simulink model "ScriptDemo"  (R2022b)
settings: configuration reference "TmVcThermal_Configuration_sub" (kept outside this file)
undefined symbols (not defined in the file or in its folder): aaaa, bbbb, cTmComprCtrl_D_u8HvacFlowTable_db, cTmComprCtrl_D_u8HvacFlowTable_sw, cTmComprCtrl_n_i16ChillCmpIMax, cTmComprCtrl_n_i16ChillCmpIMin, cTmComprCtrl_n_i16ChillCmpIMin666, cTmComprCtrl_n_i16ChillCmpPMax, cTmComprCtrl_n_i16ChillCmpPMin, cTmComprCtrl_n_i16CmpChillCoolRpmKiMax, cTmComprCtrl_n_i16CmpChillCoolRpmKiMin, cTmComprCtrl_n_i16CmpChillCoolRpmKpMax, cTmComprCtrl_n_i16CmpChillCoolRpmKpMin, cTmComprCtrl_n_i16CmpCoolRpmKiMax, cTmComprCtrl_n_i16CmpCoolRpmKiMin, cTmComprCtrl_n_i16CmpCoolRpmKpMax, cTmComprCtrl_n_i16CmpCoolRpmKpMin, cTmComprCtrl_n_i16SM4CmpHeatKiMax, cTmComprCtrl_n_i16SM4CmpHeatKiMin, cTmComprCtrl_n_i16SM4CmpHeatKpMax, cTmComprCtrl_n_i16SM4CmpHeatKpMin, cTmComprCtrl_n_i16SM5CmpHeatKiMax, cTmComprCtrl_n_i16SM5CmpHeatKiMin, cTmComprCtrl_n_i16SM5CmpHeatKpMax, cTmComprCtrl_n_i16SM5CmpHeatKpMin, cTmComprCtrl_n_i16SM6CmpHeatKiMax, cTmComprCtrl_n_i16SM6CmpHeatKiMin, cTmComprCtrl_n_i16SM6CmpHeatKpMax, cTmComprCtrl_n_i16SM6CmpHeatKpMin, cTmComprCtrl_n_u16CmpMaxSpdFanFltLimt, cTmComprCtrl_n_u16CmpMaxSpdLoSidePFltLimt, cTmComprCtrl_n_u16CmpMaxSpdSensorFltLimt, cTmComprCtrl_n_u16CompMinRpm, cTmComprCtrl_n_u16CompRpmIncThres, cTmComprCtrl_t_u16BattCooltFFPeriod, cTmComprCtrl_t_u16BattCooltPIPeriod, cTmComprCtrl_t_u16CmpCoolFFPeriod, cTmComprCtrl_t_u16CmpCoolPIPeriod, cTmComprCtrl_t_u16CoolCmpChillFFPeriod, cTmComprCtrl_t_u16CoolCmpChillPIPeriod, cTmComprCtrl_t_u16SM4CmpHeatFFPeriod, cTmComprCtrl_t_u16SM4CmpHeatPIPeriod, cTmComprCtrl_t_u16SM5CmpHeatFFPeriod, cTmComprCtrl_t_u16SM5CmpHeatPIPeriod, cTmComprCtrl_t_u16SM6CmpHeatFFPeriod, cTmComprCtrl_t_u16SM6CmpHeatPIPeriod, cTmComprCtrl_Te_EvapClearInteg, cTmComprCtrl_Te_i16HpReqTempSaturoffset, cTmComprCtrl_Te_i16SatLpReplaceDiff, cTmComprCtrl_Te_i16SM3BatDiffStartEvapDecOffset, cTmComprCtrl_Te_i16SM3EvapLo, cTmComprCtrl_Te_i16SM3TBatDiffEntEvapDecOffset, cTmComprCtrl_Te_i16SM3TBatDiffEntEvapDecOffsetQuit, cTmComprCtrl_Te_s32ErrCmpChillPIContinueCoolH, cTmComprCtrl_Te_s32ErrCmpChillPIContinueCoolL, cTmComprCtrl_Te_s32ErrCmpPIContinueChillH, cTmComprCtrl_Te_s32ErrCmpPIContinueChillL, cTmComprCtrl_Te_s32ErrCmpPIContinueCoolH, cTmComprCtrl_Te_s32ErrCmpPIContinueCoolL, cTmComprCtrl_Te_s32ErrCmpPIContinueHeatH ... (+398)
libraries: simulink x846, PCMULib x711, simulink_need_slupdate x4
(part 5 of 49)

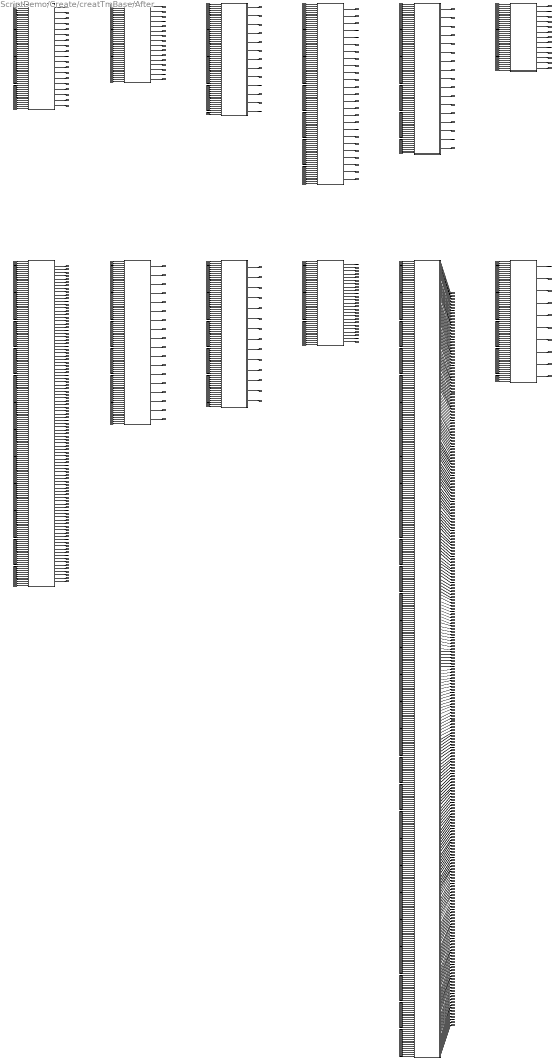
== system ScriptDemo/Create/creatTmBase/After ==
  TmAfCtrl : ModelReference  ModelNameDialog=TmAfCtrl  ScheduleRates=on  ModelReferenceVersion=13.542
  TmColtModeMgr : ModelReference  ModelNameDialog=TmColtModeMgr  ScheduleRates=on  ModelReferenceVersion=3.463
  TmColtVlvCtrl : ModelReference  ModelNameDialog=TmColtVlvCtrl  ScheduleRates=on  ModelReferenceVersion=1.683
  TmComprCtrl : ModelReference  ModelNameDialog=TmComprCtrl  ScheduleRates=on  ModelReferenceVersion=1.3185
  TmDiag : ModelReference  ModelNameDialog=TmDiag  ScheduleRates=on  ModelReferenceVersion=13.625
  TmEnergyMgr : ModelReference  ModelNameDialog=TmEnergyMgr  ScheduleRates=on  ModelReferenceVersion=1.192
  TmHvchCtrl : ModelReference  ModelNameDialog=TmHvchCtrl  ScheduleRates=on  ModelReferenceVersion=3.667
  TmPumpCtrl : ModelReference  ModelNameDialog=TmPumpCtrl  ScheduleRates=on  ModelReferenceVersion=1.672
  TmRefriModeMgr : ModelReference  ModelNameDialog=TmRefriModeMgr  ScheduleRates=on  ModelReferenceVersion=6.965
  TmRefriVlvCtrl : ModelReference  ModelNameDialog=TmRefriVlvCtrl  ScheduleRates=on  ModelReferenceVersion=1.1331
  TmSigProces : ModelReference  ModelNameDialog=TmSigProces  ScheduleRates=on  ModelReferenceVersion=1.556
  TmSovCtrl : ModelReference  ModelNameDialog=TmSovCtrl  ScheduleRates=on  ModelReferenceVersion=1.508
  wires:
  [TmRefriModeMgr_100] -> TmRefriModeMgr/1
  [yTmIn_B_AirCondEnbl] -> TmRefriModeMgr/2
  [yTmIn_B_HvacHeatgReq] -> TmRefriModeMgr/3
  [sTmIn_D_u8HvacFanSts] -> TmRefriModeMgr/4
  [sTmSigProces_Te_s32TAmb] -> TmRefriModeMgr/5
  [sTmSigProces_Te_s32HvBattCooltTOutFilter] -> TmRefriModeMgr/6
  [sTmSigProces_Te_s32BattHvMinFilter] -> TmRefriModeMgr/7
  [sTmSigProces_Te_s32EvapFanReqRamp] -> TmRefriModeMgr/8
  [sTmSigProces_Te_s32HeatrAirTReqRamp] -> TmRefriModeMgr/9
  [sTmSigProces_Te_s32HvBattCooltTFilter] -> TmRefriModeMgr/10
  [sTmDiag_D_u8BattPmpFltSt] -> TmRefriModeMgr/11
  [sTmSigProces_D_u8PowerFault] -> TmRefriModeMgr/12
  [yTmIn_B_CPSRFbSt] -> TmRefriModeMgr/13
  [sTmIn_D_u8HvActvSts] -> TmRefriModeMgr/14
  [sTmSigProces_D_u8BattThermReq] -> TmRefriModeMgr/15
  [sTmDiag_D_u8RefriMod2FInhitReq] -> TmRefriModeMgr/16
  [sTmIn_X_s32BexvPosSts] -> TmRefriModeMgr/17
  [sTmIn_n_s32ElacCmprActl] -> TmRefriModeMgr/18
  [sTmSigProces_D_u8HeatPumpConfig] -> TmRefriModeMgr/19
  [sTmComprCtrl_n_u16CompMaxRpm] -> TmRefriModeMgr/20
  [sTmSigProces_Te_s32HvacHexAirTFilter] -> TmRefriModeMgr/21
  [sTmSigProces_D_u8TempDualFlag] -> TmRefriModeMgr/22
  [sTmIn_Pw_s32HvHeatrPwrCns] -> TmRefriModeMgr/23
  [sTmColtModeMgr_D_u8WSMCurMode] -> TmRefriModeMgr/24
  [sTmSigProces_Te_s32SatLp] -> TmRefriModeMgr/25
  [sTmSigProces_md_u16BlwCool] -> TmRefriModeMgr/26
  [sTmSigProces_p_u16PLowSide] -> TmRefriModeMgr/27
  [sTmSigProces_Pw_i16ReqPwrForHeat] -> TmRefriModeMgr/28
  [sTmSigProces_Te_s32EvapFanFilter] -> TmRefriModeMgr/29
  [sTmSigProces_Te_s32TempInlet] -> TmRefriModeMgr/30
  [yTmHvchCtrl_B_HpcPtcEnad] -> TmRefriModeMgr/31
  [sTmRefriVlvCtrl_Z_u8BEXVInitState] -> TmRefriModeMgr/32
  [sTmRefriVlvCtrl_Z_u8EEXVInitState] -> TmRefriModeMgr/33
  [sTmRefriVlvCtrl_Z_u8CEXVInitState] -> TmRefriModeMgr/34
  [sTmComprCtrl_D_u8CmprRefriSwitchSt] -> TmRefriModeMgr/35
  [sTmRefriVlvCtrl_D_u8EexvRefriSwitchSt] -> TmRefriModeMgr/36
  [sTmRefriVlvCtrl_D_u8CexvRefriSwitchSt] -> TmRefriModeMgr/37
  [sTmRefriVlvCtrl_D_u8BexvRefriSwitchSt] -> TmRefriModeMgr/38
  [sTmSovCtrl_D_u8SOV1RefriSwitchSt] -> TmRefriModeMgr/39
  [sTmSovCtrl_D_u8SOV2RefriSwitchSt] -> TmRefriModeMgr/40
  [sTmSovCtrl_D_u8SOV3RefriSwitchSt] -> TmRefriModeMgr/41
  [sTmSigProces_D_u8CarChrgMode] -> TmRefriModeMgr/42
  [sTmIn_Te_s32HvBattCooltTReq] -> TmRefriModeMgr/43
  [yTmComprCtrl_B_CompOnReq] -> TmRefriModeMgr/44
  [sTmSigProces_Te_s32SatHp] -> TmRefriModeMgr/45
  [sTmIn_Te_s32WtrTInOutl] -> TmRefriModeMgr/46
  [sTmSigProces_Te_s32BattHvMaxFilter] -> TmRefriModeMgr/47
  [sTmIn_X_s32BctvPosSts] -> TmRefriModeMgr/48
  [sTmSigProces_md_u16BlwHeat] -> TmRefriModeMgr/49
  [yTmIn_B_EcoClimaSts] -> TmRefriModeMgr/50
  [sTmIn_D_u8UsgModSts1WdSts] -> TmRefriModeMgr/51
  [sTmIn_X_s32ClimtRcirc] -> TmRefriModeMgr/52
  [sTmColtModeMgr_B_HvBattClntHtgHvac] -> TmRefriModeMgr/53
  [sTmIn_Te_s32HvBattTAvg] -> TmRefriModeMgr/54
  [sTmHvchCtrl_Te_s32CabinPtcTempReq] -> TmRefriModeMgr/55
  TmRefriModeMgr/1 -> [sTmRefriModeMgr_D_u8CabinCoolReq]
  TmRefriModeMgr/2 -> [sTmRefriModeMgr_D_u8CabinHeatReq]
  TmRefriModeMgr/3 -> [sTmRefriModeMgr_D_u8BatCoolReq]
  TmRefriModeMgr/4 -> [sTmRefriModeMgr_D_u8HPAbleToWHRFlag]
  TmRefriModeMgr/5 -> [sTmRefriModeMgr_D_u8ModeStatus]
  TmRefriModeMgr/6 -> [sTmRefriModeMgr_D_u8HPCurMode]
  TmRefriModeMgr/7 -> [sTmRefriModeMgr_D_u8HpModeMainState]
  TmRefriModeMgr/8 -> [sTmRefriModeMgr_D_u8HpModeCmd]
  TmRefriModeMgr/9 -> [sTmRefriModeMgr_D_u8HpFmCmd]
  TmRefriModeMgr/10 -> [sTmRefriModeMgr_D_u8HpReqPTCState]
  TmRefriModeMgr/11 -> [yTmRefriModeMgr_B_InterChillDeicing]
  TmRefriModeMgr/12 -> [yTmRefriModeMgr_B_DeicePTCReq]
  TmRefriModeMgr/13 -> [yTmRefriModeMgr_B_CoolOCRMode]
  TmRefriModeMgr/14 -> [yTmRefriModeMgr_B_NeedPTCInOCR]
  TmRefriModeMgr/15 -> [yTmRefriModeMgr_B_CoolModeInCycle]
  TmRefriModeMgr/16 -> [sTmRefriModeMgr_D_u8ModeSwitchType]
  TmRefriModeMgr/17 -> [sTmRefriModeMgr_D_u8HvacMixClapOpenReq]
  TmRefriModeMgr/18 -> [yTmRefriModeMgr_B_HpReqPTCAddHeat]
  TmRefriModeMgr/19 -> [yTmRefriModeMgr_B_HeatModeInCycle]
  [TmColtModeMgr_100] -> TmColtModeMgr/1
  [yTmIn_B_CPSRFbSt] -> TmColtModeMgr/2
  [sTmSigProces_D_u8PowerFault] -> TmColtModeMgr/3
  [yTmRefriModeMgr_B_InterChillDeicing] -> TmColtModeMgr/4
  [sTmDiag_D_u8BctvFltSt] -> TmColtModeMgr/5
  [sTmDiag_D_u8BcfvFltSt] -> TmColtModeMgr/6
  [sTmDiag_D_u8ClntTforEmCircFltSt] -> TmColtModeMgr/7
  [sTmDiag_D_u8EmPmpFltSt] -> TmColtModeMgr/8
  [sTmDiag_D_u8BattPmpFltSt] -> TmColtModeMgr/9
  [sTmIn_D_u8HvActvSts] -> TmColtModeMgr/10
  [sTmDiag_D_u8WaterMod2FInhitReq] -> TmColtModeMgr/11
  [sTmSigProces_D_u8BattThermReq] -> TmColtModeMgr/12
  [sTmIn_v_s32VehSpdLgt] -> TmColtModeMgr/13
  [sTmSigProces_Te_s32MotorCoolt] -> TmColtModeMgr/14
  [sTmSigProces_Te_s32BattHvMaxFilter] -> TmColtModeMgr/15
  [sTmSigProces_Te_s32BattHvMinFilter] -> TmColtModeMgr/16
  [sTmSigProces_D_u8PassiveCoolEnFlag] -> TmColtModeMgr/17
  [sTmSigProces_Te_s32HvBattCooltTOutFilter] -> TmColtModeMgr/18
  [yTmRefriModeMgr_B_NeedPTCInOCR] -> TmColtModeMgr/19
  [yTmRefriModeMgr_B_CoolOCRMode] -> TmColtModeMgr/20
  [sTmSigProces_Te_s32HeatrAirTReqRamp] -> TmColtModeMgr/21
  [sTmIn_X_s32BcfvPosSts] -> TmColtModeMgr/22
  [sTmIn_X_s32BctvPosSts] -> TmColtModeMgr/23
  [sTmIn_D_u8HeatPump] -> TmColtModeMgr/24
  [sTmSigProces_Te_s32TAmb] -> TmColtModeMgr/25
  [sTmIn_Te_s32HvBattTAvg] -> TmColtModeMgr/26
  [sTmRefriModeMgr_D_u8CabinHeatReq] -> TmColtModeMgr/27
  [sTmSigProces_Te_s32HvBattCooltTFilter] -> TmColtModeMgr/28
  [yTmRefriModeMgr_B_DeicePTCReq] -> TmColtModeMgr/29
  [sTmIn_D_u8HeatStopReq] -> TmColtModeMgr/30
  [yTmHvchCtrl_B_EdMoterHeatEnad] -> TmColtModeMgr/31
  [sTmComprCtrl_D_u32AcOffCode] -> TmColtModeMgr/32
  [sTmComprCtrl_D_u32AcOffCode2] -> TmColtModeMgr/33
  [sTmEnergyMgr_Pw_s32HvCoolgPwrNormDes] -> TmColtModeMgr/34
  [sTmIn_Pw_s32HvCoolgAllwd] -> TmColtModeMgr/35
  [sTmIn_Pw_s32HvHeatgAllwd] -> TmColtModeMgr/36
  [sTmHvchCtrl_D_u32PtcOffCode] -> TmColtModeMgr/37
  [sTmEnergyMgr_Pw_s32HvHeatgPwrNormDes] -> TmColtModeMgr/38
  [yTmRefriModeMgr_B_HeatModeInCycle] -> TmColtModeMgr/39
  [sTmIn_D_u8UsgModSts1WdSts] -> TmColtModeMgr/40
  [sTmRefriModeMgr_D_u8HpReqPTCState] -> TmColtModeMgr/41
  TmColtModeMgr/1 -> [sTmColtModeMgr_D_u8WSMSwitchState]
  TmColtModeMgr/2 -> [sTmColtModeMgr_D_u8WSMCurMode]
  TmColtModeMgr/3 -> [sTmColtModeMgr_D_u8WSMReqModeFront]
  TmColtModeMgr/4 -> [yTmColtModeMgr_B_BatReqForDeiceFlag]
  TmColtModeMgr/5 -> [sTmColtModeMgr_D_u8BatReqPTCState]
  TmColtModeMgr/6 -> [sTmColtModeMgr_D_u8WaterMainState]
  TmColtModeMgr/7 -> [sTmColtModeMgr_D_u8WSMReqMode]
  TmColtModeMgr/8 -> [sTmColtModeMgr_B_HvBattClntHtgHvac]
  TmColtModeMgr/9 -> [yTmColtModeMgr_B_HeatSave]
  TmColtModeMgr/10 -> [yTmColtModeMgr_B_HvEMotorBattClntHtgHvac]
  TmColtModeMgr/11 -> [yTmColtModeMgr_B_DeiceBattAddHeat]
  TmColtModeMgr/12 -> [yTmColtModeMgr_B_NeedPTCInOCR]
  TmColtModeMgr/13 -> [yTmColtModeMgr_B_EMoterHeatModEnad]
  TmColtModeMgr/14 -> [sTmColtModeMgr_D_u8WSMFunction]
  TmColtModeMgr/15 -> [yTmColtModeMgr_B_EMoterHeatModSave]
  TmColtModeMgr/16 -> [sTmColtModeMgr_D_u8HvBattThermReqFb]
  [TmHvchCtrl_100] -> TmHvchCtrl/1
  [sTmColtModeMgr_D_u8BatReqPTCState] -> TmHvchCtrl/2
  [sTmRefriModeMgr_D_u8HpReqPTCState] -> TmHvchCtrl/3
  [yTmColtModeMgr_B_DeiceBattAddHeat] -> TmHvchCtrl/4
  [yTmRefriModeMgr_B_NeedPTCInOCR] -> TmHvchCtrl/5
  [sTmDiag_D_u8WaterMod2FInhitReq] -> TmHvchCtrl/6
  [yTmIn_B_CPSRFbSt] -> TmHvchCtrl/7
  [sTmSigProces_D_u8PowerFault] -> TmHvchCtrl/8
  [sTmIn_D_u8HeatStopReq] -> TmHvchCtrl/9
  [sTmIn_D_u8HvActvSts] -> TmHvchCtrl/10
  [yTmIn_B_HvCooltHeatrEnad] -> TmHvchCtrl/11
  [sTmDiag_D_u8HvchFltSt] -> TmHvchCtrl/12
  [sTmDiag_D_u8HmPmpFltSt] -> TmHvchCtrl/13
  [sTmDiag_D_u8BattClntLvlFltSt] -> TmHvchCtrl/14
  [sTmDiag_D_u8BctvFltSt] -> TmHvchCtrl/15
  [sTmPumpCtrl_X_s32HpumpPwmReq] -> TmHvchCtrl/16
  [sTmSigProces_Te_s32HeatrAirTReqRamp] -> TmHvchCtrl/17
  [sTmIn_Te_s32HvBattCooltTReq] -> TmHvchCtrl/18
  [sTmIn_Te_s32HvacHexAirT] -> TmHvchCtrl/19
  [sTmSigProces_Te_s32TAmb] -> TmHvchCtrl/20
  [yTmIn_B_HvacHexAirTQf] -> TmHvchCtrl/21
  [sTmIn_Te_s32HvBattCooltT] -> TmHvchCtrl/22
  [sTmIn_Te_s32WtrTInIntk] -> TmHvchCtrl/23
  [sTmIn_Te_s32WtrTInOutl] -> TmHvchCtrl/24
  [sTmColtModeMgr_B_HvBattClntHtgHvac] -> TmHvchCtrl/25
  [sTmDiag_D_u8BattPmpFltSt] -> TmHvchCtrl/26
  [sTmSigProces_D_u8BattThermReq] -> TmHvchCtrl/27
  [sTmIn_X_s32BctvPosSts] -> TmHvchCtrl/28
  [sTmSigProces_md_u16BlwHeat] -> TmHvchCtrl/29
  [sTmDiag_D_u8HvBattCooltTFltSt] -> TmHvchCtrl/30
  [sTmDiag_D_u8HvBattCooltTOutFltSt] -> TmHvchCtrl/31
  [yTmIn_B_ImpactDetect] -> TmHvchCtrl/32
  [sTmIn_D_u8HeatrStsSig] -> TmHvchCtrl/33
  [yTmIn_B_EmActivHeatAllwd] -> TmHvchCtrl/34
  [sTmSigProces_D_u8HeatPumpConfig] -> TmHvchCtrl/35
  [sTmSigProces_D_u8ElecDrivelineConfig] -> TmHvchCtrl/36
  [sTmIn_D_u8IsgHeatFdBck] -> TmHvchCtrl/37
  [sTmIn_D_u8WhlMotSysHeatFdBck] -> TmHvchCtrl/38
  [sTmIn_Pw_s32IsgHeatPwrMax] -> TmHvchCtrl/39
  [sTmIn_Pw_s32WhlMotSysHeatPwrMax] -> TmHvchCtrl/40
  [sTmSigProces_Te_s32HvBattCooltTFilter] -> TmHvchCtrl/41
  [sTmIn_Pw_s32IsgHeatPwrAct] -> TmHvchCtrl/42
  [sTmIn_Pw_s32WhlMotSysHeatPwrAct] -> TmHvchCtrl/43
  [sTmSigProces_D_u8CarChrgMode] -> TmHvchCtrl/44
  [sTmSigProces_Te_s32BattHvMinFilter] -> TmHvchCtrl/45
  [sTmEnergyMgr_Pw_s32ElecDrvHeatgPwrAllwd] -> TmHvchCtrl/46
  [sTmIn_X_s32BattCooltPmpPwmFb] -> TmHvchCtrl/47
  [sTmDiag_D_u8ClntTforEmCircFltSt] -> TmHvchCtrl/48
  [yTmRefriModeMgr_B_HpReqPTCAddHeat] -> TmHvchCtrl/49
  [sTmSigProces_Te_s32EvapFanFilter] -> TmHvchCtrl/50
  [yTmColtModeMgr_B_HvEMotorBattClntHtgHvac] -> TmHvchCtrl/51
  [sTmIn_D_u8HeatPump] -> TmHvchCtrl/52
  [sTmIn_D_u8OnBdChrgrHndlSts] -> TmHvchCtrl/53
  [sTmRefriModeMgr_D_u8CabinHeatReq] -> TmHvchCtrl/54
  [sTmDiag_Te_s32PtcTReq2F] -> TmHvchCtrl/55
  [sTmDiag_D_u8PtcT2FEnaState] -> TmHvchCtrl/56
  [yTmDiag_B_PtcEnaReq2F] -> TmHvchCtrl/57
  [sTmDiag_D_u8PtcEna2FEnaState] -> TmHvchCtrl/58
  TmHvchCtrl/1 -> [yTmHvchCtrl_B_HPumpPtcStopOk]
  TmHvchCtrl/2 -> [sTmHvchCtrl_Te_s32HpcPtcTempReq]
  TmHvchCtrl/3 -> [yTmHvchCtrl_B_HpcPtcEnad]
  TmHvchCtrl/4 -> [yTmHvchCtrl_B_HvWtrHeatrActDischrgReq]
  TmHvchCtrl/5 -> [sTmHvchCtrl_D_u32PtcOffCode]
  TmHvchCtrl/6 -> [yTmHvchCtrl_B_FrntHeatModEnad]
  TmHvchCtrl/7 -> [yTmHvchCtrl_B_RearHeatModEnad]
  TmHvchCtrl/8 -> [sTmHvchCtrl_Pw_s32ElecDrvHeatgPwrReq]
  TmHvchCtrl/9 -> [sTmHvchCtrl_Pw_u16FrntHeatPwrAllwd]
  TmHvchCtrl/10 -> [sTmHvchCtrl_Pw_u16RearHeatPwrAllwd]
  TmHvchCtrl/11 -> [yTmHvchCtrl_B_EdMoterHeatEnad]
  TmHvchCtrl/12 -> [sTmHvchCtrl_Te_s32CabinPtcTempReq]
  TmHvchCtrl/13 -> [sTmHvchCtrl_D_u8PTCOffState]
  [TmComprCtrl_100] -> TmComprCtrl/1
  [sTmDiag_D_u8BexvFltSt] -> TmComprCtrl/2
  [sTmDiag_D_u8CexvFltSt] -> TmComprCtrl/3
  [sTmDiag_D_u8EexvFltSt] -> TmComprCtrl/4
  [sTmDiag_D_u8FanFltSt] -> TmComprCtrl/5
  [sTmDiag_D_u8HiSidePFltSt] -> TmComprCtrl/6
  [sTmDiag_D_u8LoSidePFltSt] -> TmComprCtrl/7
  [sTmDiag_D_u8OutrCondOutTFltSt] -> TmComprCtrl/8
  [sTmDiag_D_u8Sov1FltSt] -> TmComprCtrl/9
  [sTmDiag_D_u8Sov2FltSt] -> TmComprCtrl/10
  [sTmDiag_D_u8Sov3FltSt] -> TmComprCtrl/11
  [sTmDiag_D_u8Sov4FltSt] -> TmComprCtrl/12
  [sTmDiag_D_u8Sov5FltSt] -> TmComprCtrl/13
  [sTmDiag_D_u8TeEvapFltSt] -> TmComprCtrl/14
  [sTmIn_D_u8DCChrgSt] -> TmComprCtrl/15
  [sTmIn_D_u8HeatPump] -> TmComprCtrl/16
  [sTmIn_D_u8HvActvSts] -> TmComprCtrl/17
  [sTmIn_I_s32ElacCmprHvActl] -> TmComprCtrl/18
  [sTmIn_Pw_s32HvCoolgAllwd] -> TmComprCtrl/19
  [sTmIn_Te_s32BattHv] -> TmComprCtrl/20
  [sTmSigProces_Te_s32EvapFanReqRamp] -> TmComprCtrl/21
  [sTmIn_Te_s32HvBattCooltT] -> TmComprCtrl/22
  [sTmIn_Te_s32HvBattCooltTReq] -> TmComprCtrl/23
  [sTmIn_U_s32ElacCmprHvActl] -> TmComprCtrl/24
  [sTmIn_X_s32BexvPosSts] -> TmComprCtrl/25
  [sTmIn_X_s32CexvPosSts] -> TmComprCtrl/26
  [sTmIn_X_s32ClimtRcirc] -> TmComprCtrl/27
  [sTmIn_X_s32EexvPosSts] -> TmComprCtrl/28
  [sTmIn_X_s32HvacTFlpActlPosnFrtRowLe] -> TmComprCtrl/29
  [sTmIn_X_s32HvacTFlpActlPosnFrtRowRi] -> TmComprCtrl/30
  [sTmIn_n_s32ElacCmprActl] -> TmComprCtrl/31
  [sTmIn_v_s32VehSpdLgt] -> TmComprCtrl/32
  [sTmRefriModeMgr_D_u8HPCurMode] -> TmComprCtrl/33
  [sTmRefriModeMgr_D_u8HpFmCmd] -> TmComprCtrl/34
  [sTmRefriModeMgr_D_u8HpModeMainState] -> TmComprCtrl/35
  [sTmRefriVlvCtrl_Z_u8BEXVInitState] -> TmComprCtrl/36
  [sTmRefriVlvCtrl_Z_u8CEXVInitState] -> TmComprCtrl/37
  [sTmRefriVlvCtrl_Z_u8EEXVInitState] -> TmComprCtrl/38
  [sTmSigProces_D_u8BattThermReq] -> TmComprCtrl/39
  [sTmSigProces_D_u8HvBattCoolgReq] -> TmComprCtrl/40
  [sTmSigProces_D_u8PowerFault] -> TmComprCtrl/41
  [sTmSigProces_Te_s32CompDischarge] -> TmComprCtrl/42
  [sTmSigProces_Te_s32EvapFanFilter] -> TmComprCtrl/43
  [sTmSigProces_Te_s32HeatrAirTReqRamp] -> TmComprCtrl/44
  [sTmSigProces_Te_s32HvBattCooltTFilter] -> TmComprCtrl/45
  [sTmSigProces_Te_s32HvBattCooltTOutFilter] -> TmComprCtrl/46
  [sTmSigProces_Te_s32HvacHexAirTFilter] -> TmComprCtrl/47
  [sTmSigProces_Te_s32TempInlet] -> TmComprCtrl/48
  [sTmSigProces_Te_s32SatHp] -> TmComprCtrl/49
  [sTmSigProces_Te_s32SatLp] -> TmComprCtrl/50
  [sTmSigProces_md_u16BlwHeat] -> TmComprCtrl/51
  [sTmSigProces_p_u16PHighSide] -> TmComprCtrl/52
  [sTmSigProces_p_u16PLowSide] -> TmComprCtrl/53
  [sTmSovCtrl_D_u8HpcSov1OnOffSts] -> TmComprCtrl/54
  [sTmSovCtrl_D_u8HpcSov2OnOffSts] -> TmComprCtrl/55
  [sTmSovCtrl_D_u8HpcSov3OnOffSts] -> TmComprCtrl/56
  [sTmSovCtrl_D_u8HpcSov4OnOffSts] -> TmComprCtrl/57
  [sTmSovCtrl_D_u8HpcSov5OnOffSts] -> TmComprCtrl/58
  [yTmHvchCtrl_B_HpcPtcEnad] -> TmComprCtrl/59
  [yTmIn_B_ElAcEnable] -> TmComprCtrl/60
  [yTmRefriModeMgr_B_CoolModeInCycle] -> TmComprCtrl/61
  [yTmSovCtrl_B_HpmSov1ActvCmd] -> TmComprCtrl/62
  [yTmSovCtrl_B_HpmSov2ActvCmd] -> TmComprCtrl/63
  [yTmSovCtrl_B_HpmSov3ActvCmd] -> TmComprCtrl/64
  [yTmSovCtrl_B_HpmSov4ActvCmd] -> TmComprCtrl/65
  [yTmSovCtrl_B_HpmSov5ActvCmd] -> TmComprCtrl/66
  [sTmDiag_D_u8AccmFltSt] -> TmComprCtrl/67
  [sTmDiag_D_u8CmprPwrEna2FEnaState] -> TmComprCtrl/68
  [sTmDiag_D_u8CmprSpdEna2FEnaState] -> TmComprCtrl/69
  [sTmDiag_D_u8CmprStsEna2FEnaState] -> TmComprCtrl/70
  [sTmDiag_D_u8CmprStsEnaReq2F] -> TmComprCtrl/71
  [sTmDiag_D_u8HiSidePNHPFltSt] -> TmComprCtrl/72
  [sTmDiag_D_u8HvacHexAirTFltSt] -> TmComprCtrl/73
  [sTmDiag_D_u8InrCondOutTFltSt] -> TmComprCtrl/74
  [sTmDiag_D_u8RefrilackFltSt] -> TmComprCtrl/75
  [sTmDiag_Pw_s32CmprPwrEnaReq2F] -> TmComprCtrl/76
  [sTmDiag_n_s32CmprSpdReq2F] -> TmComprCtrl/77
  [sTmDiag_D_u8CmprDischrgTFltSt] -> TmComprCtrl/78
  [sTmSigProces_Pw_i16ReqPwrForHeat] -> TmComprCtrl/79
  [sTmSigProces_md_u16BlwCool] -> TmComprCtrl/80
  [sTmSigProces_D_u8CarChrgMode] -> TmComprCtrl/81
  [sTmIn_D_u8ElecDriveline] -> TmComprCtrl/82
  [sTmRefriModeMgr_D_u8CabinCoolReq] -> TmComprCtrl/83
  [sTmRefriModeMgr_D_u8CabinHeatReq] -> TmComprCtrl/84
  [sTmRefriModeMgr_D_u8HpModeCmd] -> TmComprCtrl/85
  [sTmSigProces_Te_s32TAmb] -> TmComprCtrl/86
  [sTmRefriModeMgr_D_u8ModeSwitchType] -> TmComprCtrl/87
  [yTmRefriModeMgr_B_CoolOCRMode] -> TmComprCtrl/88
  [sTmDiag_D_u8BattPmpFltSt] -> TmComprCtrl/89
  [sTmDiag_D_u8HvBattCooltTFltSt] -> TmComprCtrl/90
  [sTmDiag_D_u8HvBattCooltTOutFltSt] -> TmComprCtrl/91
  [sTmIn_D_u8OnBdChrgrHndlSts] -> TmComprCtrl/92
  [sTmSigProces_Pw_i16ReqPwrForCool] -> TmComprCtrl/93
  [yTmRefriModeMgr_B_HeatModeInCycle] -> TmComprCtrl/94
  TmComprCtrl/1 -> [sTmComprCtrl_D_u32AcOffCode]
  TmComprCtrl/2 -> [sTmComprCtrl_n_u16CompRpmReq]
  TmComprCtrl/3 -> [yTmComprCtrl_B_CompOnReq]
  TmComprCtrl/4 -> [sTmComprCtrl_n_u16CompMaxRpm]
  TmComprCtrl/5 -> [sTmComprCtrl_D_u8AcOffCode0]
  TmComprCtrl/6 -> [sTmComprCtrl_D_u8AcOffCode1]
  TmComprCtrl/7 -> [sTmComprCtrl_D_u8AcOffCode2]
  TmComprCtrl/8 -> [sTmComprCtrl_D_u8AcOffCode3]
  TmComprCtrl/9 -> [sTmComprCtrl_D_u8AirCondCmpsrStats]
  TmComprCtrl/10 -> [sTmComprCtrl_Pw_s32ClimaCoolgPwrCritDes]
  TmComprCtrl/11 -> [sTmComprCtrl_Pw_s32CmprPwrNormDes]
  TmComprCtrl/12 -> [sTmComprCtrl_Pw_s32CoolgPwrCritDes]
  TmComprCtrl/13 -> [sTmComprCtrl_Pw_s32ElacCmprMax]
  TmComprCtrl/14 -> [sTmComprCtrl_Pw_s32HpcHvCoolgPwrCns]
  TmComprCtrl/15 -> [sTmComprCtrl_X_u8HpcCoolgLoad]
  TmComprCtrl/16 -> [sTmComprCtrl_t_u32CmprRunTime]
  TmComprCtrl/17 -> [yTmComprCtrl_B_AcPHiSideHi]
  TmComprCtrl/18 -> [yTmComprCtrl_B_AcPLoSideLo]
  TmComprCtrl/19 -> [yTmComprCtrl_B_HpcCoolgLimd]
  TmComprCtrl/20 -> [yTmComprCtrl_B_AcPHiSideLo]
  TmComprCtrl/21 -> [sTmComprCtrl_D_u32AcOffCode2]
  TmComprCtrl/22 -> [sTmComprCtrl_D_u8AcOffCode4]
  TmComprCtrl/23 -> [sTmComprCtrl_D_u8HvacFlowLevel]
  TmComprCtrl/24 -> [sTmComprCtrl_D_u8CmprRefriSwitchSt]
  TmComprCtrl/25 -> [sTmComprCtrl_D_u8ACOffState]
  [TmRefriVlvCtrl_100] -> TmRefriVlvCtrl/1
  [sTmComprCtrl_D_u8CmprRefriSwitchSt] -> TmRefriVlvCtrl/2
  [sTmComprCtrl_D_u8HvacFlowLevel] -> TmRefriVlvCtrl/3
  [sTmComprCtrl_n_u16CompMaxRpm] -> TmRefriVlvCtrl/4
  [sTmComprCtrl_n_u16CompRpmReq] -> TmRefriVlvCtrl/5
  [sTmDiag_D_u8BexvCal2FEnaState] -> TmRefriVlvCtrl/6
  [sTmDiag_D_u8BexvFltSt] -> TmRefriVlvCtrl/7
  [sTmDiag_D_u8BexvMoveEna2FEnaState] -> TmRefriVlvCtrl/8
  [sTmDiag_D_u8BexvPosnReq2FEnaState] -> TmRefriVlvCtrl/9
  [sTmDiag_D_u8CexvCal2FEnaState] -> TmRefriVlvCtrl/10
  [sTmDiag_D_u8CexvFltSt] -> TmRefriVlvCtrl/11
  [sTmDiag_D_u8CexvMoveEna2FEnaState] -> TmRefriVlvCtrl/12
  [sTmDiag_D_u8CexvPosnReq2FEnaState] -> TmRefriVlvCtrl/13
  [sTmDiag_D_u8ChillerOutTFltSt] -> TmRefriVlvCtrl/14
  [sTmDiag_D_u8EexvCal2FEnaState] -> TmRefriVlvCtrl/15
  [sTmDiag_D_u8EexvFltSt] -> TmRefriVlvCtrl/16
  [sTmDiag_D_u8EexvMoveEna2FEnaState] -> TmRefriVlvCtrl/17
  [sTmDiag_D_u8EexvPosnReq2FEnaState] -> TmRefriVlvCtrl/18
  [sTmDiag_D_u8EvapOutTFltSt] -> TmRefriVlvCtrl/19
  [sTmDiag_D_u8HiSidePFltSt] -> TmRefriVlvCtrl/20
  [sTmDiag_D_u8InrCondOutTFltSt] -> TmRefriVlvCtrl/21
  [sTmDiag_D_u8LoSidePFltSt] -> TmRefriVlvCtrl/22
  [sTmDiag_D_u8OutrCondOutTFltSt] -> TmRefriVlvCtrl/23
  [sTmDiag_X_s32BexvPosnReq2F] -> TmRefriVlvCtrl/24
  [sTmDiag_X_s32CexvPosnReq2F] -> TmRefriVlvCtrl/25
  [sTmDiag_X_s32EexvPosnReq2F] -> TmRefriVlvCtrl/26
  [sTmIn_D_u8BexvCalibSts] -> TmRefriVlvCtrl/27
  [sTmIn_D_u8CexvCalibSts] -> TmRefriVlvCtrl/28
  [sTmIn_D_u8EexvCalibSts] -> TmRefriVlvCtrl/29
  [sTmIn_D_u8HeatPump] -> TmRefriVlvCtrl/30
  [sTmIn_D_u8HvBattCoolgReq] -> TmRefriVlvCtrl/31
  [sTmIn_L_s32HvBattCoolFlow1] -> TmRefriVlvCtrl/32
  [sTmIn_Te_s32HvBattCooltTReq] -> TmRefriVlvCtrl/33
  [sTmIn_X_s32BexvPosSts] -> TmRefriVlvCtrl/34
  [sTmIn_X_s32CexvPosSts] -> TmRefriVlvCtrl/35
  [sTmIn_X_s32EexvPosSts] -> TmRefriVlvCtrl/36
  [sTmIn_v_s32VehSpdLgt] -> TmRefriVlvCtrl/37
  [sTmRefriModeMgr_D_u8HPCurMode] -> TmRefriVlvCtrl/38
  [sTmRefriModeMgr_D_u8HpModeCmd] -> TmRefriVlvCtrl/39
  [sTmRefriModeMgr_D_u8HpModeMainState] -> TmRefriVlvCtrl/40
  [sTmRefriModeMgr_D_u8HpReqPTCState] -> TmRefriVlvCtrl/41
  [sTmRefriModeMgr_D_u8ModeSwitchType] -> TmRefriVlvCtrl/42
  [sTmSigProces_D_u8CarChrgMode] -> TmRefriVlvCtrl/43
  [sTmSigProces_D_u8LargerCoolingFlag] -> TmRefriVlvCtrl/44
  [sTmSigProces_Pw_i16ReqPwrForCool] -> TmRefriVlvCtrl/45
  [sTmSigProces_Te_s32BattHvMaxFilter] -> TmRefriVlvCtrl/46
  [sTmSigProces_Te_s32CompDischarge] -> TmRefriVlvCtrl/47
  [sTmSigProces_Te_s32CoolSH] -> TmRefriVlvCtrl/48
  [sTmSigProces_Te_s32CurInterSC] -> TmRefriVlvCtrl/49
  [sTmSigProces_Te_s32CurOutSC] -> TmRefriVlvCtrl/50
  [sTmSigProces_Te_s32CurSCCalValue] -> TmRefriVlvCtrl/51
  [sTmSigProces_Te_s32EvapFanFilter] -> TmRefriVlvCtrl/52
  [sTmSigProces_Te_s32EvapFanReqRamp] -> TmRefriVlvCtrl/53
  [sTmSigProces_Te_s32HeatSH] -> TmRefriVlvCtrl/54
  [sTmSigProces_Te_s32HeatrAirTReqRamp] -> TmRefriVlvCtrl/55
  [sTmSigProces_Te_s32HvBattCooltTFilter] -> TmRefriVlvCtrl/56
  [sTmSigProces_Te_s32HvBattCooltTOutFilter] -> TmRefriVlvCtrl/57
  [sTmSigProces_Te_s32HvacHexAirTFilter] -> TmRefriVlvCtrl/58
  [sTmSigProces_Te_s32InletCal] -> TmRefriVlvCtrl/59
  [sTmSigProces_Te_s32TAmb] -> TmRefriVlvCtrl/60
  [sTmSigProces_md_u16BlwCool] -> TmRefriVlvCtrl/61
  [sTmSigProces_md_u16BlwHeat] -> TmRefriVlvCtrl/62
  [sTmSigProces_p_u16PHighSide] -> TmRefriVlvCtrl/63
  [sTmSigProces_p_u16PLowSide] -> TmRefriVlvCtrl/64
  [sTmSovCtrl_D_u8SOV2RefriSwitchSt] -> TmRefriVlvCtrl/65
  [yTmComprCtrl_B_CompOnReq] -> TmRefriVlvCtrl/66
  [yTmDiag_B_BexvCalReq2F] -> TmRefriVlvCtrl/67
  [yTmDiag_B_BexvMoveEnReq2F] -> TmRefriVlvCtrl/68
  [yTmDiag_B_CexvCalReq2F] -> TmRefriVlvCtrl/69
  [yTmDiag_B_CexvMoveEnReq2F] -> TmRefriVlvCtrl/70
  [yTmDiag_B_EexvCalReq2F] -> TmRefriVlvCtrl/71
  [yTmDiag_B_EexvMoveEnReq2F] -> TmRefriVlvCtrl/72
  [yTmHvchCtrl_B_HpcPtcEnad] -> TmRefriVlvCtrl/73
  [yTmIn_B_CPSRFbSt] -> TmRefriVlvCtrl/74
  [yTmIn_B_HmiMaxACReq] -> TmRefriVlvCtrl/75
  [yTmRefriModeMgr_B_CoolModeInCycle] -> TmRefriVlvCtrl/76
  [yTmRefriModeMgr_B_CoolOCRMode] -> TmRefriVlvCtrl/77
  [yTmRefriModeMgr_B_InterChillDeicing] -> TmRefriVlvCtrl/78
  TmRefriVlvCtrl/1 -> [yTmRefriVlvCtrl_B_HpcCexvMovEnable]
  TmRefriVlvCtrl/2 -> [yTmRefriVlvCtrl_B_CexvCalibReq]
  TmRefriVlvCtrl/3 -> [yTmRefriVlvCtrl_B_HpcEexvMovEnable]
  TmRefriVlvCtrl/4 -> [yTmRefriVlvCtrl_B_EexvCalibReq]
  TmRefriVlvCtrl/5 -> [yTmRefriVlvCtrl_B_HpcBexvMovEnable]
  TmRefriVlvCtrl/6 -> [yTmRefriVlvCtrl_B_BexvCalibReq]
  TmRefriVlvCtrl/7 -> [sTmRefriVlvCtrl_X_s32SM3BexvMaxPos]
  TmRefriVlvCtrl/8 -> [yTmRefriVlvCtrl_B_EvapBattTLimBexvEna]
  TmRefriVlvCtrl/9 -> [sTmRefriVlvCtrl_D_u8EexvRefriSwitchSt]
  TmRefriVlvCtrl/10 -> [sTmRefriVlvCtrl_D_u8CexvRefriSwitchSt]
  TmRefriVlvCtrl/11 -> [sTmRefriVlvCtrl_D_u8BexvRefriSwitchSt]
  TmRefriVlvCtrl/12 -> [sTmRefriVlvCtrl_X_s32EEXVPosReq]
  TmRefriVlvCtrl/13 -> [sTmRefriVlvCtrl_Z_u8CEXVInitState]
  TmRefriVlvCtrl/14 -> [sTmRefriVlvCtrl_Z_u8EEXVInitState]
  TmRefriVlvCtrl/15 -> [sTmRefriVlvCtrl_Z_u8BEXVInitState]
  TmRefriVlvCtrl/16 -> [sTmRefriVlvCtrl_X_s32CEXVPosReq]
  TmRefriVlvCtrl/17 -> [sTmRefriVlvCtrl_X_s32BEXVPosReq]
  [TmSovCtrl_100] -> TmSovCtrl/1
  [sTmRefriModeMgr_D_u8HpModeMainState] -> TmSovCtrl/2
  [sTmDiag_D_u8ChillerValve2FEnState] -> TmSovCtrl/3
  [sTmDiag_D_u8EvaprVlvFrnt2FEnState] -> TmSovCtrl/4
  [sTmDiag_D_u8HpmSov1Actv2FEnState] -> TmSovCtrl/5
  [sTmDiag_D_u8HpmSov2Actv2FEnState] -> TmSovCtrl/6
  [sTmDiag_D_u8HpmSov3Actv2FEnState] -> TmSovCtrl/7
  [yTmDiag_B_ChillerValveReq2F] -> TmSovCtrl/8
  [yTmDiag_B_EvaprVlvReqFrnt2F] -> TmSovCtrl/9
  [yTmDiag_B_HpmSov1ActvCmd2F] -> TmSovCtrl/10
  [yTmDiag_B_HpmSov2ActvCmd2F] -> TmSovCtrl/11
  [yTmDiag_B_HpmSov3ActvCmd2F] -> TmSovCtrl/12
  [sTmComprCtrl_D_u8CmprRefriSwitchSt] -> TmSovCtrl/13
  [sTmRefriModeMgr_D_u8ModeSwitchType] -> TmSovCtrl/14
  [sTmRefriVlvCtrl_D_u8BexvRefriSwitchSt] -> TmSovCtrl/15
  [sTmRefriVlvCtrl_D_u8CexvRefriSwitchSt] -> TmSovCtrl/16
  [sTmRefriVlvCtrl_D_u8EexvRefriSwitchSt] -> TmSovCtrl/17
  [yTmIn_B_ChillerValveReqFb] -> TmSovCtrl/18
  [yTmIn_B_EvaprVlvReqFrntFb] -> TmSovCtrl/19
  [yTmIn_B_HpmSov1ActvCmdFb] -> TmSovCtrl/20
  [yTmIn_B_HpmSov2ActvCmdFb] -> TmSovCtrl/21
  [yTmIn_B_HpmSov3ActvCmdFb] -> TmSovCtrl/22
  [sTmIn_D_u8DCChrgSt] -> TmSovCtrl/23
  [sTmIn_Te_s32HvBattCooltT] -> TmSovCtrl/24
  [sTmIn_Te_s32HvBattCooltTReq] -> TmSovCtrl/25
  [sTmPumpCtrl_L_s32BpumpFlwEstmd] -> TmSovCtrl/26
  [sTmSigProces_Te_s32BattHvMaxFilter] -> TmSovCtrl/27
  [sTmSigProces_D_u8BattThermReq] -> TmSovCtrl/28
  [sTmSigProces_md_u16BlwCool] -> TmSovCtrl/29
  [sTmSigProces_p_u16PHighSide] -> TmSovCtrl/30
  [yTmComprCtrl_B_CompOnReq] -> TmSovCtrl/31
  [yTmIn_B_AirCondEnbl] -> TmSovCtrl/32
  [sTmSigProces_Te_s32HvBattCooltTFilter] -> TmSovCtrl/33
  [sTmSigProces_Te_s32EvapFanFilter] -> TmSovCtrl/34
  [yTmRefriModeMgr_B_CoolModeInCycle] -> TmSovCtrl/35
  TmSovCtrl/1 -> [yTmSovCtrl_B_HpmSov1ActvCmd]
  TmSovCtrl/2 -> [yTmSovCtrl_B_HpmSov2ActvCmd]
  TmSovCtrl/3 -> [yTmSovCtrl_B_HpmSov3ActvCmd]
  TmSovCtrl/4 -> [yTmSovCtrl_B_HpmSov4ActvCmd]
  TmSovCtrl/5 -> [yTmSovCtrl_B_HpmSov5ActvCmd]
  TmSovCtrl/6 -> [sTmSovCtrl_D_u8HpcSov1OnOffSts]
  TmSovCtrl/7 -> [sTmSovCtrl_D_u8HpcSov2OnOffSts]
  TmSovCtrl/8 -> [sTmSovCtrl_D_u8HpcSov3OnOffSts]
  TmSovCtrl/9 -> [sTmSovCtrl_D_u8HpcSov4OnOffSts]
  TmSovCtrl/10 -> [sTmSovCtrl_D_u8HpcSov5OnOffSts]
  TmSovCtrl/11 -> [sTmSovCtrl_D_u8SOV1RefriSwitchSt]
  TmSovCtrl/12 -> [sTmSovCtrl_D_u8SOV2RefriSwitchSt]
  TmSovCtrl/13 -> [sTmSovCtrl_D_u8SOV3RefriSwitchSt]
  [TmSigProces_100] -> TmSigProces/1
  [sTmIn_D_u8DistHvBatt] -> TmSigProces/2
  [sTmIn_D_u8ElecDriveline] -> TmSigProces/3
  [sTmIn_D_u8CruiseCtrl] -> TmSigProces/4
  [sTmIn_D_u8Refrigerant] -> TmSigProces/5
  [sTmIn_D_u8HeatPump] -> TmSigProces/6
  [sTmIn_D_u8HiWayAsst] -> TmSigProces/7
  [sTmIn_D_u8HvBoostMod] -> TmSigProces/8
  [sTmDiag_D_u8HiSidePFltSt] -> TmSigProces/9
  [sTmIn_U_s32HiSideP] -> TmSigProces/10
  [sTmDiag_D_u8LoSidePFltSt] -> TmSigProces/11
  [sTmIn_U_s32LoSideP] -> TmSigProces/12
  [sTmDiag_D_u8OutrCondOutTFltSt] -> TmSigProces/13
  [sTmIn_U_s32AcIntelCondOutT] -> TmSigProces/14
  [sTmDiag_D_u8ChillerOutTFltSt] -> TmSigProces/15
  [sTmIn_U_s32AcCompInletT] -> TmSigProces/16
  [sTmDiag_D_u8EvapOutTFltSt] -> TmSigProces/17
  [sTmIn_U_s32AcEvapOutT] -> TmSigProces/18
  [sTmDiag_D_u8CmprDischrgTFltSt] -> TmSigProces/19
  [sTmIn_U_s32AcCompDischrgT] -> TmSigProces/20
  [sTmDiag_D_u8InrCondOutTFltSt] -> TmSigProces/21
  [sTmIn_U_s32AcCondOutT] -> TmSigProces/22
  [sTmDiag_D_u8ClntTforEmCircFltSt] -> TmSigProces/23
  [sTmIn_U_s32CooltTSigForDtElec] -> TmSigProces/24
  [sTmIn_Te_s32AmbTEstimd] -> TmSigProces/25
  [yTmIn_B_AmbTEstimdQf] -> TmSigProces/26
  [sTmIn_Te_s32IncarTemp] -> TmSigProces/27
  [sTmIn_D_u8IncarTempQf] -> TmSigProces/28
  [sTmIn_Te_s32HvBattCooltTReq] -> TmSigProces/29
  [sTmIn_Te_s32HvBattCooltT] -> TmSigProces/30
  [sTmIn_Te_s32HvBattCooltTOut] -> TmSigProces/31
  [sTmIn_Te_s32BattHvMin] -> TmSigProces/32
  [sTmIn_Te_s32BattHv] -> TmSigProces/33
  [sTmIn_Te_s32OnBdChrgrCooltT] -> TmSigProces/34
  [sTmIn_Te_s32Coolt] -> TmSigProces/35
  [sTmIn_Te_s32WhlMotSysCooltT] -> TmSigProces/36
  [sTmIn_v_s32VehSpdLgt] -> TmSigProces/37
  [sTmIn_Te_s32Evap] -> TmSigProces/38
  [yTmIn_B_TeEvap] -> TmSigProces/39
  [sTmIn_Te_s32EvapReq] -> TmSigProces/40
  [sTmIn_Te_s32WtrTInOutl] -> TmSigProces/41
  [sTmIn_md_s32HvacAirMFlowEstimd] -> TmSigProces/42
  [sTmIn_D_u8HvacFanSts] -> TmSigProces/43
  [sTmIn_md_s32HexHeatrAirMFlowEstimd] -> TmSigProces/44
  [sTmIn_D_u8DCChrgSt] -> TmSigProces/45
  [sTmIn_D_u8OnBdChrgrHndlSts] -> TmSigProces/46
  [sTmIn_X_s32ClimtRcirc] -> TmSigProces/47
  [sTmIn_X_s32HvacTFlpActlPosnFrtRowLe] -> TmSigProces/48
  [sTmIn_X_s32HvacTFlpActlPosnFrtRowRi] -> TmSigProces/49
  [sTmIn_Te_s32HmiCmptmtTSpForRowFirstLe] -> TmSigProces/50
  [sTmIn_Te_s32HmiCmptmtTSpForRowFirstRi] -> TmSigProces/51
  [sTmIn_D_u8SysQf] -> TmSigProces/52
  [sTmIn_U_s32Sys] -> TmSigProces/53
  [yTmIn_B_CPSRFbSt] -> TmSigProces/54
  [sTmIn_D_u8BcfvFaultSts] -> TmSigProces/55
  [sTmIn_D_u8BcfvVoltSts] -> TmSigProces/56
  [sTmDiag_D_u8BcfvFltSt] -> TmSigProces/57
  [sTmIn_D_u8BctvFaultSts] -> TmSigProces/58
  [sTmIn_D_u8BctvVoltSts] -> TmSigProces/59
  [sTmDiag_D_u8BctvFltSt] -> TmSigProces/60
  [sTmIn_D_u8BexvElecStsErr] -> TmSigProces/61
  [sTmIn_D_u8BexvBlkErr] -> TmSigProces/62
  [sTmDiag_D_u8BexvFltSt] -> TmSigProces/63
  [sTmIn_D_u8BexvOvrTempErr] -> TmSigProces/64
  [sTmIn_D_u8BexvVoltgRangErr] -> TmSigProces/65
  [sTmIn_D_u8CexvElecStsErr] -> TmSigProces/66
  [sTmDiag_D_u8CexvFltSt] -> TmSigProces/67
  [sTmIn_D_u8CexvBlkErr] -> TmSigProces/68
  [sTmIn_D_u8CexvOvrTempErr] -> TmSigProces/69
  [sTmIn_D_u8CexvVoltgRangErr] -> TmSigProces/70
  [sTmDiag_D_u8AgmFltSt] -> TmSigProces/71
  [sTmDiag_D_u8BattPmpFltSt] -> TmSigProces/72
  [sTmDiag_D_u8EmPmpFltSt] -> TmSigProces/73
  [sTmDiag_D_u8FanFltSt] -> TmSigProces/74
  [sTmDiag_D_u8HmPmpFltSt] -> TmSigProces/75
  [sTmIn_D_u8EctvFaultSts] -> TmSigProces/76
  [sTmDiag_D_u8EctvFltSt] -> TmSigProces/77
  [sTmIn_D_u8EctvVoltSts] -> TmSigProces/78
  [sTmIn_D_u8EexvBlkErr] -> TmSigProces/79
  [sTmIn_D_u8EexvElecStsErr] -> TmSigProces/80
  [sTmIn_D_u8EexvOvrTempErr] -> TmSigProces/81
  [sTmIn_D_u8EexvVoltgRangErr] -> TmSigProces/82
  [sTmDiag_D_u8EexvFltSt] -> TmSigProces/83
  [sTmIn_D_u8HvBattCooltLvl] -> TmSigProces/84
  [sTmIn_D_u8HVoltResonanceStat] -> TmSigProces/85
  [sTmIn_D_u8InCurrOverCurrStat] -> TmSigProces/86
  [sTmIn_D_u8MotorCurrOverCurrStat] -> TmSigProces/87
  [sTmIn_D_u8OverMotorCurrStat] -> TmSigProces/88
  [sTmIn_D_u8CmprRotorLockStat] -> TmSigProces/89
  [yTmIn_B_EvaprTFrntUD] -> TmSigProces/90
  [yTmIn_B_HvacHexAirTUD] -> TmSigProces/91
  [sTmDiag_D_u8Sov3FltSt] -> TmSigProces/92
  [sTmDiag_D_u8Sov2FltSt] -> TmSigProces/93
  [sTmDiag_D_u8Sov1FltSt] -> TmSigProces/94
  [sTmIn_D_u8SelfTmpSigHwProtn] -> TmSigProces/95
  [sTmIn_D_u8CooltTInSnsrFlt] -> TmSigProces/96
  [sTmIn_D_u8CooltTOutSnsrFlt] -> TmSigProces/97
  [sTmIn_D_u8TInMtrlSnsrFlt] -> TmSigProces/98
  [sTmIn_D_u8CircForDrvrShoOrOpen] -> TmSigProces/99
  [sTmIn_D_u8ICnsOutOfRng] -> TmSigProces/100
  [sTmIn_D_u8MemErr] -> TmSigProces/101
  [sTmIn_D_u8CooltTOutOfRng] -> TmSigProces/102
  [sTmIn_D_u8FltInComHVCH] -> TmSigProces/103
  [sTmIn_D_u8HvOutOfRng] -> TmSigProces/104
  [sTmIn_D_u8ULoOutOfRng] -> TmSigProces/105
  [sTmDiag_D_u8HvchFltSt] -> TmSigProces/106
  [sTmDiag_D_u8HpmSov1Actv2FEnState] -> TmSigProces/107
  [sTmDiag_D_u8HpmSov2Actv2FEnState] -> TmSigProces/108
  [sTmDiag_D_u8HpmSov3Actv2FEnState] -> TmSigProces/109
  [sTmDiag_D_u8BexvPosnReq2FEnaState] -> TmSigProces/110
  [sTmDiag_D_u8BexvCal2FEnaState] -> TmSigProces/111
  [sTmDiag_D_u8BexvMoveEna2FEnaState] -> TmSigProces/112
  [sTmDiag_D_u8CexvPosnReq2FEnaState] -> TmSigProces/113
  [sTmDiag_D_u8CexvCal2FEnaState] -> TmSigProces/114
  [sTmDiag_D_u8CexvMoveEna2FEnaState] -> TmSigProces/115
  [sTmDiag_D_u8EexvPosnReq2FEnaState] -> TmSigProces/116
  [sTmDiag_D_u8EexvCal2FEnaState] -> TmSigProces/117
  [sTmDiag_D_u8EexvMoveEna2FEnaState] -> TmSigProces/118
  [sTmDiag_D_u8CmprPwrEna2FEnaState] -> TmSigProces/119
  [sTmDiag_D_u8CmprStsEna2FEnaState] -> TmSigProces/120
  [sTmDiag_D_u8CmprSpdEna2FEnaState] -> TmSigProces/121
  [sTmDiag_D_u8PTCPumpSpd2FEnState] -> TmSigProces/122
  [sTmDiag_D_u8EmCooltPmp2FEnState] -> TmSigProces/123
  [sTmDiag_D_u8BattCooltPmp2FEnState] -> TmSigProces/124
  [sTmDiag_D_u8PtcPwr2FEnaState] -> TmSigProces/125
  [sTmDiag_D_u8PtcT2FEnaState] -> TmSigProces/126
  [sTmDiag_D_u8PtcEna2FEnaState] -> TmSigProces/127
  [sTmDiag_D_u8BctvVlvPos2FEnaState] -> TmSigProces/128
  [sTmDiag_D_u8BctvVlvRef2FEnaState] -> TmSigProces/129
  [sTmDiag_D_u8BcfvVlvPos2FEnaState] -> TmSigProces/130
  [sTmDiag_D_u8BcfvVlvRef2FEnaState] -> TmSigProces/131
  [sTmDiag_D_u8EctvVlvPos2FEnaState] -> TmSigProces/132
  [sTmDiag_D_u8EctvVlvMoveEna2FEnaState] -> TmSigProces/133
  [sTmIn_D_u8LnchModSts] -> TmSigProces/134
  [sTmIn_D_u8LaunchCtrl] -> TmSigProces/135
  [sTmDiag_D_u8HiSidePNHPFltSt] -> TmSigProces/136
  [sTmRefriModeMgr_D_u8HpReqPTCState] -> TmSigProces/137
  [yTmRefriModeMgr_B_DeicePTCReq] -> TmSigProces/138
  [sTmRefriModeMgr_D_u8HpModeCmd] -> TmSigProces/139
  [sTmColtModeMgr_D_u8WSMReqMode] -> TmSigProces/140
  [sTmColtModeMgr_D_u8WSMCurMode] -> TmSigProces/141
  [sTmRefriVlvCtrl_Z_u8CEXVInitState] -> TmSigProces/142
  [sTmRefriVlvCtrl_Z_u8EEXVInitState] -> TmSigProces/143
  [sTmRefriVlvCtrl_Z_u8BEXVInitState] -> TmSigProces/144
  [sTmIn_U_s32HiSidePNHP] -> TmSigProces/145
  [sTmIn_Te_s32HvacHexAirT] -> TmSigProces/146
  [yTmIn_B_HvacHexAirTQf] -> TmSigProces/147
  [sTmIn_Te_s32HeatrAirTReq] -> TmSigProces/148
  [sTmIn_D_u8HvActvSts] -> TmSigProces/149
  [sTmIn_D_u8HvBattThermReq] -> TmSigProces/150
  [sTmIn_D_u8HvBattCoolgReq] -> TmSigProces/151
  [sTmIn_D_u8HvBattHeatgReq] -> TmSigProces/152
  [sTmRefriModeMgr_D_u8HPCurMode] -> TmSigProces/153
  [sTmRefriModeMgr_D_u8CabinHeatReq] -> TmSigProces/154
  [sTmDiag_D_u8HvBattCooltTFltSt] -> TmSigProces/155
  [sTmPumpCtrl_L_s32BpumpFlwEstmd] -> TmSigProces/156
  [sTmDiag_D_u8TeEvapFltSt] -> TmSigProces/157
  [sTmRefriModeMgr_D_u8CabinCoolReq] -> TmSigProces/158
  [sTmPumpCtrl_X_s32MpumpPwmReq] -> TmSigProces/159
  [sTmDiag_D_u8HvBattCooltTOutFltSt] -> TmSigProces/160
  [sTmDiag_D_u8HvacHexAirTFltSt] -> TmSigProces/161
  [sTmIn_D_u16HVvBattLimnIndcn] -> TmSigProces/162
  [sTmIn_D_u8SrvRqrdResd] -> TmSigProces/163
  [yTmIn_B_HmiMaxACReq] -> TmSigProces/164
  [yTmPumpCtrl_B_MpumpCpsrReq] -> TmSigProces/165
  [sTmIn_n_s32ElacCmprActl] -> TmSigProces/166
  [sTmIn_Te_s32TDcDcCoolt] -> TmSigProces/167
  [yTmDiag_B_HvBattLimnIndcnUDLost] -> TmSigProces/168
  [yTmHvchCtrl_B_HvWtrHeatrActDischrgReq] -> TmSigProces/169
  TmSigProces/1 -> [sTmSigProces_D_u8AdcuConfig]
  TmSigProces/2 -> [sTmSigProces_p_u16PHighSide]
  TmSigProces/3 -> [sTmSigProces_p_s32HpAcHiSidePToOut]
  TmSigProces/4 -> [sTmSigProces_p_u16PLowSide]
  TmSigProces/5 -> [sTmSigProces_p_s32LoSideToOut]
  TmSigProces/6 -> [sTmSigProces_Te_s32HighSide]
  TmSigProces/7 -> [sTmSigProces_Te_s32AcIntelCondOutToOut]
  TmSigProces/8 -> [sTmSigProces_Te_s32CompInlet]
  TmSigProces/9 -> [sTmSigProces_Te_s32AcCompInletToOut]
  TmSigProces/10 -> [sTmSigProces_Te_s32EvapOut]
  TmSigProces/11 -> [sTmSigProces_Te_s32AcEvapOutToOut]
  TmSigProces/12 -> [sTmSigProces_Te_s32CompDischarge]
  TmSigProces/13 -> [sTmSigProces_Te_s32AcCompDischrgToOut]
  TmSigProces/14 -> [sTmSigProces_Te_s32InteCondOutlet]
  TmSigProces/15 -> [sTmSigProces_Te_s32AcCondOutToOut]
  TmSigProces/16 -> [sTmSigProces_Te_s32MotorCoolt]
  TmSigProces/17 -> [sTmSigProces_Te_s32CooltTSigForDtElecToOut]
  TmSigProces/18 -> [sTmSigProces_p_u16PHighSideNHP]
  TmSigProces/19 -> [sTmSigProces_Te_s32TAmb]
  TmSigProces/20 -> [sTmSigProces_Te_s32Incar]
  TmSigProces/21 -> [sTmSigProces_Te_s32HvBattCooltTFilter]
  TmSigProces/22 -> [sTmSigProces_Te_s32HvBattCooltTOutFilter]
  TmSigProces/23 -> [sTmSigProces_Te_s32BattHvMinFilter]
  TmSigProces/24 -> [sTmSigProces_Te_s32BattHvMaxFilter]
  TmSigProces/25 -> [sTmSigProces_Te_s32MotorDvcCtl]
  TmSigProces/26 -> [sTmSigProces_md_s32EFanMaxFow]
  TmSigProces/27 -> [sTmSigProces_Te_s32EvapFanFilter]
  TmSigProces/28 -> [sTmSigProces_Te_s32EvapFanReqRamp]
  TmSigProces/29 -> [sTmSigProces_Te_s32HvacHexAirTFilter]
  TmSigProces/30 -> [sTmSigProces_Te_s32HeatrAirTReqRamp]
  TmSigProces/31 -> [sTmSigProces_Te_s32SatHp]
  TmSigProces/32 -> [sTmSigProces_Te_s32SatLp]
  TmSigProces/33 -> [sTmSigProces_Te_s32CurSC]
  TmSigProces/34 -> [sTmSigProces_Te_s32CurSCCalValue]
  TmSigProces/35 -> [sTmSigProces_Te_s32CoolSH]
  TmSigProces/36 -> [sTmSigProces_Te_s32HeatSH]
  TmSigProces/37 -> [sTmSigProces_Te_s32CurDischargeSH]
  TmSigProces/38 -> [sTmSigProces_Te_s32HvacHexAirTEstimd]
  TmSigProces/39 -> [sTmSigProces_Te_s32AirTFromHeatgEstimdToOut]
  TmSigProces/40 -> [sTmSigProces_md_u16BlwCool]
  TmSigProces/41 -> [sTmSigProces_md_u16BlwHeat]
  TmSigProces/42 -> [sTmSigProces_D_u8CarChrgMode]
  TmSigProces/43 -> [sTmSigProces_Pw_i16ReqPwrForHeat]
  TmSigProces/44 -> [sTmSigProces_Te_s32InletCal]
  TmSigProces/45 -> [sTmSigProces_D_u8TempDualFlag]
  TmSigProces/46 -> [sTmSigProces_D_u8BattThermReq]
  TmSigProces/47 -> [sTmSigProces_D_u8PowerFault]
  TmSigProces/48 -> [sTmSigProces_D_u8PassiveCoolEnFlag]
  TmSigProces/49 -> [sTmSigProces_Z_u8Fault_LoSideT]
  TmSigProces/50 -> [sTmSigProces_Z_u8Fault_HiSidePT]
  TmSigProces/51 -> [yTmSigProces_B_Fault_DischrgT]
  TmSigProces/52 -> [sTmSigProces_Z_u8Fault_EvapOut]
  TmSigProces/53 -> [yTmSigProces_B_Fault_EvapT]
  TmSigProces/54 -> [yTmSigProces_B_Fault_HexT]
  TmSigProces/55 -> [yTmSigProces_B_Fault_CmpInlet]
  TmSigProces/56 -> [yTmSigProces_B_Fault_SOV1]
  TmSigProces/57 -> [sTmSigProces_Z_u8Fault_SOV2]
  TmSigProces/58 -> [yTmSigProces_B_Fault_SOV2Cmp]
  TmSigProces/59 -> [yTmSigProces_B_Fault_SOV3]
  TmSigProces/60 -> [sTmSigProces_Z_u8Fault_Cexv]
  TmSigProces/61 -> [sTmSigProces_Z_u8Fault_Eexv]
  TmSigProces/62 -> [sTmSigProces_Z_u8Fault_Bexv]
  TmSigProces/63 -> [sTmSigProces_Z_u8Fault_Fan]
  TmSigProces/64 -> [yTmSigProces_B_Fault_CmpSelf]
  TmSigProces/65 -> [yTmSigProces_B_Fault_Ectv]
  TmSigProces/66 -> [yTmSigProces_B_Fault_Bctv]
  TmSigProces/67 -> [yTmSigProces_B_Fault_Bcfv]
  TmSigProces/68 -> [yTmSigProces_B_Fault_TMotor]
  TmSigProces/69 -> [sTmSigProces_Z_u8Fault_BatLvl]
  TmSigProces/70 -> [yTmSigProces_B_Fault_PtcSelf]
  TmSigProces/71 -> [sTmSigProces_Z_u8Fault_HPump]
  TmSigProces/72 -> [sTmSigProces_Z_u8Fault_BPump]
  TmSigProces/73 -> [sTmSigProces_Z_u8Fault_MPump]
  TmSigProces/74 -> [yTmSigProces_B_Fault_Ags]
  TmSigProces/75 -> [yTmSigProces_B_Hp2FCtrlEnable]
  TmSigProces/76 -> [yTmSigProces_B_Wm2FCtrlEnable]
  TmSigProces/77 -> [sTmSigProces_D_u8MaxCoolingTestFlag]
  TmSigProces/78 -> [yTmSigProces_B_LaunchCtrl]
  TmSigProces/79 -> [sTmSigProces_Te_s32condReqOffectIncMC]
  TmSigProces/80 -> [sTmSigProces_Te_s32condReqOffectIncMC2]
  TmSigProces/81 -> [sTmSigProces_p_s32HiSidePNHPToOut]
  TmSigProces/82 -> [sTmSigProces_Te_s32TempInlet]
  TmSigProces/83 -> [sTmSigProces_Te_s32CurInterSC]
  TmSigProces/84 -> [sTmSigProces_Te_s32CurOutSC]
  TmSigProces/85 -> [sTmSigProces_D_u8HvBattCoolgReq]
  TmSigProces/86 -> [sTmSigProces_D_u8HvBattHeatgReq]
  TmSigProces/87 -> [sTmSigProces_D_u8DistHvBattConfig]
  TmSigProces/88 -> [sTmSigProces_D_u8ElecDrivelineConfig]
  TmSigProces/89 -> [sTmSigProces_D_u8CruiseCtrlConfig]
  TmSigProces/90 -> [sTmSigProces_D_u8RefrigerantConfig]
  TmSigProces/91 -> [sTmSigProces_D_u8HeatPumpConfig]
  TmSigProces/92 -> [sTmSigProces_D_u8HiWayAsstConfig]
  TmSigProces/93 -> [sTmSigProces_D_u8HvBoostModConfig]
  TmSigProces/94 -> [sTmSigProces_D_u8LargerCoolingFlag]
  TmSigProces/95 -> [yTmSigProces_B_CpsrRlyFrmClima]
  TmSigProces/96 -> [sTmSigProces_D_u8LaunchCtrlConfig]
  TmSigProces/97 -> [sTmSigProces_D_u8PTCSupplier]
  TmSigProces/98 -> [sTmSigProces_Pw_i16ReqPwrForCool]
  TmSigProces/99 -> [sTmSigProces_D_u16HVvBattLimnIndcn]
  [TmPumpCtrl_100] -> TmPumpCtrl/1
  [sTmIn_L_s32OnBdChrgrMinCooltFlow] -> TmPumpCtrl/2
  [sTmIn_L_s32DcDcMinCooltFlow] -> TmPumpCtrl/3
  [sTmIn_L_s32IsgCooltFlowMinReq] -> TmPumpCtrl/4
  [sTmIn_L_s32WhlMotCooltFlowMinReq] -> TmPumpCtrl/5
  [sTmIn_Te_s32EradWndgActl] -> TmPumpCtrl/6
  [sTmIn_D_u8OnBdChrgrHndlSts] -> TmPumpCtrl/7
  [sTmIn_Te_s32HvgWndgActl] -> TmPumpCtrl/8
  [sTmDiag_D_u8EmPmpFltSt] -> TmPumpCtrl/9
  [yTmDiag_B_CarConfigInvalid] -> TmPumpCtrl/10
  [yTmSigProces_B_LaunchCtrl] -> TmPumpCtrl/11
  [sTmIn_D_u8HvActvSts] -> TmPumpCtrl/12
  [yTmIn_B_CPSRFbSt] -> TmPumpCtrl/13
  [sTmIn_D_u8PowerPackStatus] -> TmPumpCtrl/14
  [sTmIn_Te_s32OnBdChrgrCooltT] -> TmPumpCtrl/15
  [sTmIn_Te_s32WhlMotSysCooltT] -> TmPumpCtrl/16
  [sTmIn_Te_s32TDcDcCoolt] -> TmPumpCtrl/17
  [sTmDiag_D_u8ClntTforEmCircFltSt] -> TmPumpCtrl/18
  [sTmIn_Te_s32Coolt] -> TmPumpCtrl/19
  [sTmIn_D_u8HvActvReq] -> TmPumpCtrl/20
  [sTmIn_Te_s32EradInvActl] -> TmPumpCtrl/21
  [sTmIn_D_u8HeatPump] -> TmPumpCtrl/22
  [sTmSigProces_Te_s32MotorCoolt] -> TmPumpCtrl/23
  [sTmDiag_D_u8EmCooltPmp2FEnState] -> TmPumpCtrl/24
  [sTmDiag_X_s32EmCooltPmpReq2F] -> TmPumpCtrl/25
  [sTmColtModeMgr_D_u8WSMCurMode] -> TmPumpCtrl/26
  [sTmIn_D_u8EctvPosSts] -> TmPumpCtrl/27
  [sTmSigProces_D_u8AdcuConfig] -> TmPumpCtrl/28
  [sTmSigProces_D_u8PowerFault] -> TmPumpCtrl/29
  [sTmIn_D_u8HvBattThermReq] -> TmPumpCtrl/30
  [sTmIn_md_s32HexHeatrAirMFlowEstimd] -> TmPumpCtrl/31
  [yTmIn_B_ImpactDetect] -> TmPumpCtrl/32
  [sTmIn_L_s32HvBattCoolFlow1] -> TmPumpCtrl/33
  [sTmColtModeMgr_B_HvBattClntHtgHvac] -> TmPumpCtrl/34
  [sTmDiag_D_u8BattPmpFltSt] -> TmPumpCtrl/35
  [sTmSigProces_D_u16HVvBattLimnIndcn] -> TmPumpCtrl/36
  [sTmDiag_D_u8BattClntLvlFltSt] -> TmPumpCtrl/37
  [sTmDiag_X_s32BattCooltPmpReq2F] -> TmPumpCtrl/38
  [sTmDiag_D_u8BattCooltPmp2FEnState] -> TmPumpCtrl/39
  [sTmSigProces_Te_s32HvBattCooltTOutFilter] -> TmPumpCtrl/40
  [sTmSigProces_D_u8CarChrgMode] -> TmPumpCtrl/41
  [yTmRefriModeMgr_B_InterChillDeicing] -> TmPumpCtrl/42
  [yTmRefriModeMgr_B_CoolModeInCycle] -> TmPumpCtrl/43
  [sTmIn_X_s32BexvPosSts] -> TmPumpCtrl/44
  [yTmRefriModeMgr_B_CoolOCRMode] -> TmPumpCtrl/45
  [sTmSigProces_Te_s32TAmb] -> TmPumpCtrl/46
  [sTmRefriModeMgr_D_u8HpReqPTCState] -> TmPumpCtrl/47
  [sTmSigProces_Te_s32HeatrAirTReqRamp] -> TmPumpCtrl/48
  [sTmIn_v_s32VehSpdLgt] -> TmPumpCtrl/49
  [sTmDiag_D_u8HmPmpFltSt] -> TmPumpCtrl/50
  [sTmIn_Te_s32WtrTInIntk] -> TmPumpCtrl/51
  [sTmColtModeMgr_D_u8BatReqPTCState] -> TmPumpCtrl/52
  [sTmRefriModeMgr_D_u8HPCurMode] -> TmPumpCtrl/53
  [sTmDiag_X_s32PTCPumpSpdReq2F] -> TmPumpCtrl/54
  [sTmDiag_D_u8PTCPumpSpd2FEnState] -> TmPumpCtrl/55
  [sTmDiag_D_u8HvchFltSt] -> TmPumpCtrl/56
  [sTmIn_U_s32Sys] -> TmPumpCtrl/57
  [sTmColtModeMgr_D_u8WaterMainState] -> TmPumpCtrl/58
  [sTmColtModeMgr_D_u8WSMSwitchState] -> TmPumpCtrl/59
  [sTmColtModeMgr_D_u8WSMReqMode] -> TmPumpCtrl/60
  [sTmIn_L_s32DHUCooltFlowMinReq] -> TmPumpCtrl/61
  [yTmIn_B_AD4CoolReq] -> TmPumpCtrl/62
  [sTmIn_D_u8ElecDriveline] -> TmPumpCtrl/63
  [sTmIn_L_s32AD4CooltFlowReq] -> TmPumpCtrl/64
  [sTmIn_D_u8HvBattCooltLvl] -> TmPumpCtrl/65
  [sTmDiag_D_u8WaterMod2FInhitReq] -> TmPumpCtrl/66
  [yTmHvchCtrl_B_HPumpPtcStopOk] -> TmPumpCtrl/67
  [sTmSigProces_D_u8BattThermReq] -> TmPumpCtrl/68
  [sTmRefriModeMgr_D_u8CabinHeatReq] -> TmPumpCtrl/69
  [sTmDiag_D_u8PtcFlow2FEnaState] -> TmPumpCtrl/70
  [sTmDiag_L_s32PtcFlowrateReq2F] -> TmPumpCtrl/71
  [sTmColtVlvCtrl_D_u8HeatgMode] -> TmPumpCtrl/72
  [yTmIn_B_AD4CoolReqForBkp] -> TmPumpCtrl/73
  [sTmIn_L_s32AD4CooltFlowReqForBkp] -> TmPumpCtrl/74
  [yTmDiag_B_AD4CooltFlowReqForBkpUDLost] -> TmPumpCtrl/75
  [yTmDiag_B_AD4CooltFlowReqUDLost] -> TmPumpCtrl/76
  [yTmDiag_B_AD4CoolReqForBkpUDLost] -> TmPumpCtrl/77
  [yTmDiag_B_AD4CoolReqUDLost] -> TmPumpCtrl/78
  [sTmIn_D_u8UsgModSts1WdSts] -> TmPumpCtrl/79
  [sTmColtModeMgr_D_u8WSMFunction] -> TmPumpCtrl/80
  [sTmRefriModeMgr_D_u8HpModeMainState] -> TmPumpCtrl/81
  [sTmRefriModeMgr_D_u8HpModeCmd] -> TmPumpCtrl/82
  [sTmIn_Te_s32HvBattTAvg] -> TmPumpCtrl/83
  [yTmHvchCtrl_B_HpcPtcEnad] -> TmPumpCtrl/84
  [sTmIn_Te_s32WtrTInOutl] -> TmPumpCtrl/85
  TmPumpCtrl/1 -> [sTmPumpCtrl_X_s32MpumpPwmReq]
  TmPumpCtrl/2 -> [sTmPumpCtrl_L_s32MpumpFlwEstmd]
  TmPumpCtrl/3 -> [sTmPumpCtrl_X_s32BpumpPwmReq]
  TmPumpCtrl/4 -> [sTmPumpCtrl_L_s32BpumpFlwEstmd]
  TmPumpCtrl/5 -> [sTmPumpCtrl_X_s32HpumpPwmReq]
  TmPumpCtrl/6 -> [sTmPumpCtrl_L_s32HpumpFlwEstmd]
  TmPumpCtrl/7 -> [yTmPumpCtrl_B_HtrPmpSpdLim]
  TmPumpCtrl/8 -> [sTmPumpCtrl_X_s32HeatrPmpPwmActTmp]
  TmPumpCtrl/9 -> [sTmPumpCtrl_n_s32HeaterPmpSpdTmp]
  TmPumpCtrl/10 -> [sTmPumpCtrl_Te_s32CooltTSigForDtElecNHP]
  TmPumpCtrl/11 -> [sTmPumpCtrl_I_s32HeatrPmpIAct]
  TmPumpCtrl/12 -> [sTmPumpCtrl_fq_s32EmCooltPmpPwmFrq]
  TmPumpCtrl/13 -> [sTmPumpCtrl_fq_s32BattCooltPmpPwmFrq]
  TmPumpCtrl/14 -> [sTmPumpCtrl_fq_s32PTCPumpPwmFrq]
  TmPumpCtrl/15 -> [sTmPumpCtrl_D_u8HPumpSubState]
  TmPumpCtrl/16 -> [yTmPumpCtrl_B_HvBattHeatOutCtrl]
  TmPumpCtrl/17 -> [yTmPumpCtrl_B_MpumpCpsrReq]
  TmPumpCtrl/18 -> [sTmPumpCtrl_L_s32MpumpFlwReq]
  [TmColtVlvCtrl_100] -> TmColtVlvCtrl/1
  [yTmRefriModeMgr_B_CoolOCRMode] -> TmColtVlvCtrl/2
  [yTmRefriModeMgr_B_NeedPTCInOCR] -> TmColtVlvCtrl/3
  [yTmRefriModeMgr_B_InterChillDeicing] -> TmColtVlvCtrl/4
  [sTmRefriModeMgr_D_u8HpReqPTCState] -> TmColtVlvCtrl/5
  [sTmSigProces_Te_s32HeatrAirTReqRamp] -> TmColtVlvCtrl/6
  [yTmColtModeMgr_B_BatReqForDeiceFlag] -> TmColtVlvCtrl/7
  [sTmIn_Te_s32WtrTInOutl] -> TmColtVlvCtrl/8
  [sTmSigProces_Te_s32HvacHexAirTFilter] -> TmColtVlvCtrl/9
  [sTmSigProces_Te_s32TAmb] -> TmColtVlvCtrl/10
  [sTmIn_X_s32BcfvPosSts] -> TmColtVlvCtrl/11
  [sTmIn_D_u8BcfvRunSts] -> TmColtVlvCtrl/12
  [sTmSigProces_D_u8PowerFault] -> TmColtVlvCtrl/13
  [sTmColtModeMgr_D_u8WSMReqMode] -> TmColtVlvCtrl/14
  [sTmSigProces_Te_s32MotorDvcCtl] -> TmColtVlvCtrl/15
  [sTmSigProces_Te_s32MotorCoolt] -> TmColtVlvCtrl/16
  [sTmSigProces_D_u8BattThermReq] -> TmColtVlvCtrl/17
  [sTmSigProces_D_u8PassiveCoolEnFlag] -> TmColtVlvCtrl/18
  [sTmRefriModeMgr_D_u8CabinCoolReq] -> TmColtVlvCtrl/19
  [sTmSigProces_Te_s32HvBattCooltTFilter] -> TmColtVlvCtrl/20
  [yTmSigProces_B_LaunchCtrl] -> TmColtVlvCtrl/21
  [sTmIn_D_u8EctvRunSts] -> TmColtVlvCtrl/22
  [sTmIn_D_u8EctvPosSts] -> TmColtVlvCtrl/23
  [sTmIn_X_s32BctvPosSts] -> TmColtVlvCtrl/24
  [sTmIn_D_u8BctvRunSts] -> TmColtVlvCtrl/25
  [sTmColtModeMgr_D_u8WSMSwitchState] -> TmColtVlvCtrl/26
  [sTmColtModeMgr_D_u8WaterMainState] -> TmColtVlvCtrl/27
  [sTmIn_D_u8HeatStopReq] -> TmColtVlvCtrl/28
  [sTmDiag_D_u8HvBattCooltTFltSt] -> TmColtVlvCtrl/29
  [sTmColtModeMgr_B_HvBattClntHtgHvac] -> TmColtVlvCtrl/30
  [sTmIn_D_u8HeatPump] -> TmColtVlvCtrl/31
  [sTmIn_Te_s32HeadEstimdFirstRow] -> TmColtVlvCtrl/32
  [sTmIn_Te_s32HmiCmptmtTSpForRowFirstRi] -> TmColtVlvCtrl/33
  [sTmIn_Te_s32HmiCmptmtTSpForRowFirstLe] -> TmColtVlvCtrl/34
  [sTmSigProces_D_u8HvBattHeatgReq] -> TmColtVlvCtrl/35
  [sTmIn_md_s32HexHeatrAirMFlowEstimd] -> TmColtVlvCtrl/36
  [yTmIn_B_HvacHeatgReq] -> TmColtVlvCtrl/37
  [sTmIn_D_u8HvacFanSts] -> TmColtVlvCtrl/38
  [yTmIn_B_ClimaDefrstSts] -> TmColtVlvCtrl/39
  [sTmDiag_D_u8HvchFltSt] -> TmColtVlvCtrl/40
  [sTmDiag_D_u8HmPmpFltSt] -> TmColtVlvCtrl/41
  [sTmDiag_D_u8BctvFltSt] -> TmColtVlvCtrl/42
  [sTmDiag_D_u8BattPmpFltSt] -> TmColtVlvCtrl/43
  [sTmIn_Te_s32HvBattCooltTReq] -> TmColtVlvCtrl/44
  [sTmIn_D_u8HvBattThermReq] -> TmColtVlvCtrl/45
  [sTmDiag_D_u8WaterMod2FInhitReq] -> TmColtVlvCtrl/46
  [sTmRefriModeMgr_D_u8CabinHeatReq] -> TmColtVlvCtrl/47
  [sTmDiag_D_u8EctvVlvPos2FEnaState] -> TmColtVlvCtrl/48
  [sTmDiag_X_u8EctvVlvPosReq2F] -> TmColtVlvCtrl/49
  [sTmDiag_D_u8EctvVlvMoveEna2FEnaState] -> TmColtVlvCtrl/50
  [yTmDiag_B_EctvVlvMoveEnaReq2F] -> TmColtVlvCtrl/51
  [sTmDiag_D_u8BctvVlvPos2FEnaState] -> TmColtVlvCtrl/52
  [sTmDiag_X_u8BctvVlvPosReq2F] -> TmColtVlvCtrl/53
  [sTmDiag_D_u8BctvVlvRef2FEnaState] -> TmColtVlvCtrl/54
  [sTmDiag_D_u8BctvVlvRefReq2F] -> TmColtVlvCtrl/55
  [sTmDiag_D_u8BcfvVlvPos2FEnaState] -> TmColtVlvCtrl/56
  [sTmDiag_X_u8BcfvVlvPosReq2F] -> TmColtVlvCtrl/57
  [sTmDiag_D_u8BcfvVlvRef2FEnaState] -> TmColtVlvCtrl/58
  [sTmDiag_D_u8BcfvVlvRefReq2F] -> TmColtVlvCtrl/59
  [sTmIn_Te_s32HvBattTAvg] -> TmColtVlvCtrl/60
  [yTmColtModeMgr_B_HeatSave] -> TmColtVlvCtrl/61
  [sTmDiag_D_u8EctvFltSt] -> TmColtVlvCtrl/62
  [yTmPumpCtrl_B_HvBattHeatOutCtrl] -> TmColtVlvCtrl/63
  [yTmColtModeMgr_B_DeiceBattAddHeat] -> TmColtVlvCtrl/64
  [sTmDiag_D_u8ClntTforEmCircFltSt] -> TmColtVlvCtrl/65
  [sTmDiag_D_u8BcfvFltSt] -> TmColtVlvCtrl/66
  [sTmDiag_D_u8EmPmpFltSt] -> TmColtVlvCtrl/67
  [yTmColtModeMgr_B_HvEMotorBattClntHtgHvac] -> TmColtVlvCtrl/68
  [sTmColtModeMgr_D_u8WSMCurMode] -> TmColtVlvCtrl/69
  [sTmSigProces_Te_s32BattHvMinFilter] -> TmColtVlvCtrl/70
  [sTmDiag_D_u8HvBattCooltTOutFltSt] -> TmColtVlvCtrl/71
  [sTmColtModeMgr_D_u8WSMFunction] -> TmColtVlvCtrl/72
  [sTmIn_D_u8HvBoostMod] -> TmColtVlvCtrl/73
  [sTmSigProces_md_u16BlwHeat] -> TmColtVlvCtrl/74
  [sTmSigProces_D_u8CarChrgMode] -> TmColtVlvCtrl/75
  [sTmIn_Te_s32HeatrAirTReq] -> TmColtVlvCtrl/76
  TmColtVlvCtrl/1 -> [sTmColtVlvCtrl_X_u8BctvPosReq]
  TmColtVlvCtrl/2 -> [sTmColtVlvCtrl_X_u8BcfvPosReq]
  TmColtVlvCtrl/3 -> [sTmColtVlvCtrl_D_u8HpcBcfvRefDrvReq]
  TmColtVlvCtrl/4 -> [sTmColtVlvCtrl_D_u8HpcBcfvSpdLvlReq]
  TmColtVlvCtrl/5 -> [sTmColtVlvCtrl_D_u8HpcBcfvActvSaveReq]
  TmColtVlvCtrl/6 -> [yTmColtVlvCtrl_B_BcfvOnTrgt]
  TmColtVlvCtrl/7 -> [yTmColtVlvCtrl_B_HpcEctvMovEna]
  TmColtVlvCtrl/8 -> [sTmColtVlvCtrl_D_u8HpcEctvReq]
  TmColtVlvCtrl/9 -> [yTmColtVlvCtrl_B_EctvOnTrgt]
  TmColtVlvCtrl/10 -> [sTmColtVlvCtrl_D_u8HpcBctvRefDrvReq]
  TmColtVlvCtrl/11 -> [sTmColtVlvCtrl_D_u8HpcBctvSpdLvlReq]
  TmColtVlvCtrl/12 -> [sTmColtVlvCtrl_D_u8HpcBctvActvSaveReq]
  TmColtVlvCtrl/13 -> [yTmColtVlvCtrl_B_BctvOnTrgt]
  TmColtVlvCtrl/14 -> [sTmColtVlvCtrl_D_u8HeatgMode]
  [TmEnergyMgr_100] -> TmEnergyMgr/1
  [sTmPumpCtrl_X_s32MpumpPwmReq] -> TmEnergyMgr/2
  [sTmPumpCtrl_X_s32BpumpPwmReq] -> TmEnergyMgr/3
  [sTmPumpCtrl_L_s32BpumpFlwEstmd] -> TmEnergyMgr/4
  [sTmPumpCtrl_X_s32HpumpPwmReq] -> TmEnergyMgr/5
  [sTmPumpCtrl_L_s32HpumpFlwEstmd] -> TmEnergyMgr/6
  [sTmIn_Pw_s32HvHeatrPwrCns] -> TmEnergyMgr/7
  [sTmIn_Pw_s32HvHeatgAllwd] -> TmEnergyMgr/8
  [sTmColtModeMgr_D_u8WSMCurMode] -> TmEnergyMgr/9
  [yTmHvchCtrl_B_HpcPtcEnad] -> TmEnergyMgr/10
  [sTmIn_Pw_s32HvHeatrPwrCnsDes] -> TmEnergyMgr/11
  [sTmSigProces_Te_s32HvBattCooltTFilter] -> TmEnergyMgr/12
  [sTmSigProces_Te_s32HvBattCooltTOutFilter] -> TmEnergyMgr/13
  [sTmIn_Te_s32WtrTInIntk] -> TmEnergyMgr/14
  [sTmIn_Te_s32WtrTInOutl] -> TmEnergyMgr/15
  [yTmComprCtrl_B_CompOnReq] -> TmEnergyMgr/16
  [sTmIn_Pw_s32HvCoolgAllwd] -> TmEnergyMgr/17
  [sTmIn_U_s32ElacCmprHvActl] -> TmEnergyMgr/18
  [sTmIn_I_s32ElacCmprHvActl] -> TmEnergyMgr/19
  [sTmSigProces_md_u16BlwCool] -> TmEnergyMgr/20
  [sTmSigProces_Te_s32EvapFanFilter] -> TmEnergyMgr/21
  [sTmSigProces_Te_s32InletCal] -> TmEnergyMgr/22
  [sTmRefriModeMgr_D_u8HpModeMainState] -> TmEnergyMgr/23
  [sTmAfCtrl_X_s32FanPwmReq] -> TmEnergyMgr/24
  [sTmDiag_D_u8PtcPwr2FEnaState] -> TmEnergyMgr/25
  [sTmDiag_Pw_s32PtcPwrReq2F] -> TmEnergyMgr/26
  [sTmSigProces_Te_s32TAmb] -> TmEnergyMgr/27
  [sTmIn_Te_s32HmiCmptmtTSpForRowFirstLe] -> TmEnergyMgr/28
  [sTmIn_Te_s32HmiCmptmtTSpForRowFirstRi] -> TmEnergyMgr/29
  [yTmIn_B_EcoClimaSts] -> TmEnergyMgr/30
  [sTmIn_D_u8ElecDriveline] -> TmEnergyMgr/31
  [sTmHvchCtrl_Pw_s32ElecDrvHeatgPwrReq] -> TmEnergyMgr/32
  [sTmIn_Pw_s32ElecDrvHeatgPwrAllwd] -> TmEnergyMgr/33
  [sTmIn_Pw_s32IsgHeatPwrAct] -> TmEnergyMgr/34
  [sTmIn_Pw_s32WhlMotSysHeatPwrAct] -> TmEnergyMgr/35
  [sTmSigProces_D_u8BattThermReq] -> TmEnergyMgr/36
  [yTmIn_B_AirCondEnbl] -> TmEnergyMgr/37
  [yTmIn_B_HvacHeatgReq] -> TmEnergyMgr/38
  [yTmIn_B_CPSRFbSt] -> TmEnergyMgr/39
  [sTmRefriModeMgr_D_u8CabinHeatReq] -> TmEnergyMgr/40
  [sTmRefriModeMgr_D_u8CabinCoolReq] -> TmEnergyMgr/41
  [sTmSigProces_md_u16BlwHeat] -> TmEnergyMgr/42
  [sTmSigProces_Te_s32HvacHexAirTFilter] -> TmEnergyMgr/43
  [sTmIn_D_u8HeatPump] -> TmEnergyMgr/44
  TmEnergyMgr/1 -> [sTmEnergyMgr_Pw_s32MpumpPwrCns]
  TmEnergyMgr/2 -> [sTmEnergyMgr_Pw_s32BpumpPwrCns]
  TmEnergyMgr/3 -> [sTmEnergyMgr_Pw_s32HpumpPwrCns]
  TmEnergyMgr/4 -> [sTmEnergyMgr_Pw_s32HvHeatgPwrCns]
  TmEnergyMgr/5 -> [sTmEnergyMgr_Pw_s32HvchPwrAllwd]
  TmEnergyMgr/6 -> [sTmEnergyMgr_Pw_s32HvHeatgPwrNormDes]
  TmEnergyMgr/7 -> [sTmEnergyMgr_Pw_s32HvHeatgPwrCritDes]
  TmEnergyMgr/8 -> [sTmEnergyMgr_Pw_s32HvClimaHeatgPwrCritDes]
  TmEnergyMgr/9 -> [sTmEnergyMgr_Pw_s32HvBattHtgPwrPreEst]
  TmEnergyMgr/10 -> [sTmEnergyMgr_Pw_s32HvCoolgPwrCritDes]
  TmEnergyMgr/11 -> [sTmEnergyMgr_Pw_s32HvClimaCoolgPwrCritDes]
  TmEnergyMgr/12 -> [sTmEnergyMgr_Pw_s32HvCoolgPwrNormDes]
  TmEnergyMgr/13 -> [sTmEnergyMgr_Pw_s32AcCmprPwrLim]
  TmEnergyMgr/14 -> [sTmEnergyMgr_Pw_s32HvCoolgPwrCns]
  TmEnergyMgr/15 -> [yTmEnergyMgr_B_AllwBattCoolOnly]
  TmEnergyMgr/16 -> [sTmEnergyMgr_Pw_s32HvCabinThermPwrCns]
  TmEnergyMgr/17 -> [sTmEnergyMgr_Pw_s32HvBattThermPwrCns]
  TmEnergyMgr/18 -> [sTmEnergyMgr_Pw_s32FanPwrCns]
  TmEnergyMgr/19 -> [sTmEnergyMgr_Pw_s32HvCoolgPwrEvap]
  TmEnergyMgr/20 -> [sTmEnergyMgr_Pw_s32HvEDActHeatgPwrNormDes]
  TmEnergyMgr/21 -> [sTmEnergyMgr_Pw_s32ElecDrvHeatgPwrAllwd]
  TmEnergyMgr/22 -> [sTmEnergyMgr_Pw_s32HvEDActHeatgPwrSumCnsVgm]
  TmEnergyMgr/23 -> [sTmEnergyMgr_Pw_s32HPCoolPACCM]
  TmEnergyMgr/24 -> [sTmEnergyMgr_Pw_s32HPHeatPACCM]
  TmEnergyMgr/25 -> [sTmEnergyMgr_Pw_s32BattCoolPACCM]
  [TmDiag_100] -> TmDiag/1
  [sTmIn_D_u8EldtCoolLelIn] -> TmDiag/2
  [sTmIn_D_u8BattCoolLelIn] -> TmDiag/3
  [sTmIn_D_u8HeatrStsSig] -> TmDiag/4
  [sTmIn_Te_s32WtrTInOutl] -> TmDiag/5
  [sTmIn_U_s32Sys] -> TmDiag/6
  [sTmIn_U_s32LoSideP] -> TmDiag/7
  [sTmIn_U_s32HiSideP] -> TmDiag/8
  [sTmIn_D_u8HeatPump] -> TmDiag/9
  [yTmIn_B_StarDiagEval] -> TmDiag/10
  [yTmIn_B_CPSRFbSt] -> TmDiag/11
  [sTmIn_D_u8UsgModSts1WdSts] -> TmDiag/12
  [sTmIn_U_s32AcIntelCondOutT] -> TmDiag/13
  [sTmIn_U_s32AcCompInletT] -> TmDiag/14
  [sTmIn_U_s32AcCondOutT] -> TmDiag/15
  [sTmIn_U_s32AcEvapOutT] -> TmDiag/16
  [sTmIn_U_s32AcCompDischrgT] -> TmDiag/17
  [sTmIn_U_s32CooltTSigForDtElec] -> TmDiag/18
  [sTmIn_Z_s32RoadIncln] -> TmDiag/19
  [sTmIn_D_u8HvBattCooltLvl] -> TmDiag/20
  [sTmIn_U_s32HiSidePNHP] -> TmDiag/21
  [yTmIn_B_Sov1SBTF] -> TmDiag/22
  [yTmIn_B_Sov1SBflg] -> TmDiag/23
  [yTmIn_B_Sov1OPTF] -> TmDiag/24
  [yTmIn_B_Sov1OPflg] -> TmDiag/25
  [yTmIn_B_HpmSov1Actv2FReq] -> TmDiag/26
  [yTmIn_B_HpmSov1ActvCmd2F] -> TmDiag/27
  [yTmIn_B_Sov2SBTF] -> TmDiag/28
  [yTmIn_B_Sov2SBflg] -> TmDiag/29
  [yTmIn_B_Sov2OPTF] -> TmDiag/30
  [yTmIn_B_Sov2OPflg] -> TmDiag/31
  [yTmIn_B_HpmSov2Actv2FReq] -> TmDiag/32
  [yTmIn_B_HpmSov2ActvCmd2F] -> TmDiag/33
  [yTmIn_B_Sov3SBTF] -> TmDiag/34
  [yTmIn_B_Sov3SBflg] -> TmDiag/35
  [yTmIn_B_Sov3OPTF] -> TmDiag/36
  [yTmIn_B_Sov3OPflg] -> TmDiag/37
  [yTmIn_B_HpmSov3Actv2FReq] -> TmDiag/38
  [yTmIn_B_HpmSov3ActvCmd2F] -> TmDiag/39
  [yTmIn_B_Sov4SBTF] -> TmDiag/40
  [yTmIn_B_Sov4SBflg] -> TmDiag/41
  [yTmIn_B_Sov4OPTF] -> TmDiag/42
  [yTmIn_B_Sov4OPflg] -> TmDiag/43
  [yTmIn_B_ChillerValve2FReq] -> TmDiag/44
  [yTmIn_B_ChillerValveReq2F] -> TmDiag/45
  [yTmIn_B_Sov5SBTF] -> TmDiag/46
  [yTmIn_B_Sov5SBflg] -> TmDiag/47
  [yTmIn_B_Sov5OPTF] -> TmDiag/48
  [yTmIn_B_Sov5OPflg] -> TmDiag/49
  [yTmIn_B_EvaprVlvFrnt2FReq] -> TmDiag/50
  [yTmIn_B_EvaprVlvReqFrnt2F] -> TmDiag/51
  [yTmIn_B_FanOutSBTF] -> TmDiag/52
  [yTmIn_B_FanOutSBflg] -> TmDiag/53
  [yTmIn_B_FanOutOPTF] -> TmDiag/54
  [yTmIn_B_FanOutOPflg] -> TmDiag/55
  [yTmIn_B_FanOutSGTF] -> TmDiag/56
  [yTmIn_B_FanOutSGflg] -> TmDiag/57
  [sTmIn_t_s32FanPwmTLow] -> TmDiag/58
  [yTmIn_B_FanTHighValid] -> TmDiag/59
  [yTmIn_B_FanTLowValid] -> TmDiag/60
  [sTmIn_t_s32FanPwmTHigh] -> TmDiag/61
  [sTmIn_D_u8VcEvSBFan] -> TmDiag/62
  [yTmIn_B_FanPwm2FReq] -> TmDiag/63
  [sTmIn_X_s32FanPwmReq2F] -> TmDiag/64
  [yTmIn_B_HmPumpSBTF] -> TmDiag/65
  [yTmIn_B_HmPumpSBflg] -> TmDiag/66
  [yTmIn_B_HmPumpOCTF] -> TmDiag/67
  [yTmIn_B_HmPumpOCflg] -> TmDiag/68
  [yTmIn_B_HmPumpSGTF] -> TmDiag/69
  [yTmIn_B_HmPumpSGflg] -> TmDiag/70
  [sTmIn_t_s32HmPumpPwmTLow] -> TmDiag/71
  [yTmIn_B_HmPumpTLowValid] -> TmDiag/72
  [sTmIn_t_s32HmPumpPwmTHigh] -> TmDiag/73
  [yTmIn_B_HmPumpTHighValid] -> TmDiag/74
  [yTmIn_B_PTCPumpSpd2FReq] -> TmDiag/75
  [sTmIn_X_s32PTCPumpSpdReq2F] -> TmDiag/76
  [yTmIn_B_BattPmpSBTF] -> TmDiag/77
  [yTmIn_B_BattPmpSBflg] -> TmDiag/78
  [yTmIn_B_BattPmpOPTF] -> TmDiag/79
  [yTmIn_B_BattPmpOPflg] -> TmDiag/80
  [yTmIn_B_BattPmpSGTF] -> TmDiag/81
  [yTmIn_B_BattPmpSGflg] -> TmDiag/82
  [sTmIn_t_s32BattPmpPwmTLow] -> TmDiag/83
  [yTmIn_B_BattPmpTLowValid] -> TmDiag/84
  [sTmIn_t_s32BattPmpPwmTHigh] -> TmDiag/85
  [yTmIn_B_BattPmpTHighValid] -> TmDiag/86
  [yTmIn_B_BattPmp2FReq] -> TmDiag/87
  [sTmIn_X_s32BattCooltPmpReq2F] -> TmDiag/88
  [yTmIn_B_EmotPmpSBTF] -> TmDiag/89
  [yTmIn_B_EmotPmpSBflg] -> TmDiag/90
  [yTmIn_B_EmotPmpOPTF] -> TmDiag/91
  [yTmIn_B_EmotPmpOPflg] -> TmDiag/92
  [yTmIn_B_EmotPmpSGTF] -> TmDiag/93
  [yTmIn_B_EmotPmpSGflg] -> TmDiag/94
  [sTmIn_t_s32EmotPmpPwmTLow] -> TmDiag/95
  [yTmIn_B_EmotPmpTLowValid] -> TmDiag/96
  [sTmIn_t_s32EmotPmpPwmTHigh] -> TmDiag/97
  [yTmIn_B_EmotPmpTHighValid] -> TmDiag/98
  [yTmIn_B_EmCooltPmp2FReq] -> TmDiag/99
  [sTmIn_X_s32EmCooltPmpReq2F] -> TmDiag/100
  [sTmIn_D_u8BctvTempSts] -> TmDiag/101
  [sTmIn_D_u8BctvVoltSts] -> TmDiag/102
  [sTmIn_D_u8BctvFaultSts] -> TmDiag/103
  [sTmIn_D_u8BctvNVMFlt] -> TmDiag/104
  [yTmIn_B_BctvVlvPos2FReq] -> TmDiag/105
  [sTmIn_X_u8BctvVlvPosReq2F] -> TmDiag/106
  [yTmIn_B_BctvVlvRef2FReq] -> TmDiag/107
  [sTmIn_D_u8BctvVlvRefReq2F] -> TmDiag/108
  [sTmIn_D_u8BcfvTempSts] -> TmDiag/109
  [sTmIn_D_u8BcfvVoltSts] -> TmDiag/110
  [sTmIn_D_u8BcfvFaultSts] -> TmDiag/111
  [sTmIn_D_u8BcfvNVMFlt] -> TmDiag/112
  [yTmIn_B_BcfvVlvPos2FReq] -> TmDiag/113
  [sTmIn_X_u8BcfvVlvPosReq2F] -> TmDiag/114
  [yTmIn_B_BcfvVlvRef2FReq] -> TmDiag/115
  [sTmIn_D_u8BcfvVlvRefReq2F] -> TmDiag/116
  [sTmIn_D_u8EctvTempSts] -> TmDiag/117
  [sTmIn_D_u8EctvVoltSts] -> TmDiag/118
  [sTmIn_D_u8EctvFaultSts] -> TmDiag/119
  [yTmIn_B_EctvVlvPos2FReq] -> TmDiag/120
  [sTmIn_X_u8EctvVlvPosReq2F] -> TmDiag/121
  [yTmIn_B_EctvVlvMoveEna2FReq] -> TmDiag/122
  [yTmIn_B_EctvVlvMoveEnaReq2F] -> TmDiag/123
  [sTmIn_D_u8BexvOvrTempErr] -> TmDiag/124
  [sTmIn_D_u8BexvVoltgRangErr] -> TmDiag/125
  [sTmIn_D_u8BexvElecStsErr] -> TmDiag/126
  [sTmIn_D_u8BexvBlkErr] -> TmDiag/127
  [sTmIn_D_u8BexvOvrTrvlErr] -> TmDiag/128
  [sTmIn_D_u8BexvNVMFlt] -> TmDiag/129
  [yTmIn_B_BExvPosn2FReq] -> TmDiag/130
  [sTmIn_X_s32BExvPosnReq2F] -> TmDiag/131
  [yTmIn_B_BExvMoveEna2FReq] -> TmDiag/132
  [yTmIn_B_BExvMoveEnReq2F] -> TmDiag/133
  [yTmIn_B_BExvCal2FReq] -> TmDiag/134
  [yTmIn_B_BExvCalReq2F] -> TmDiag/135
  [sTmIn_D_u8CexvOvrTempErr] -> TmDiag/136
  [sTmIn_D_u8CexvVoltgRangErr] -> TmDiag/137
  [sTmIn_D_u8CexvElecStsErr] -> TmDiag/138
  [sTmIn_D_u8CexvBlkErr] -> TmDiag/139
  [sTmIn_D_u8CexvOvrTrvlErr] -> TmDiag/140
  [sTmIn_D_u8CexvNVMFlt] -> TmDiag/141
  [yTmIn_B_CExvPosn2FReq] -> TmDiag/142
  [sTmIn_X_s32CExvPosnReq2F] -> TmDiag/143
  [yTmIn_B_CExvMoveEna2FReq] -> TmDiag/144
  [yTmIn_B_CExvMoveEnaReq2F] -> TmDiag/145
  [yTmIn_B_CExvCal2FReq] -> TmDiag/146
  [yTmIn_B_CExvCalReq2F] -> TmDiag/147
  [sTmIn_D_u8EexvOvrTempErr] -> TmDiag/148
  [sTmIn_D_u8EexvVoltgRangErr] -> TmDiag/149
  [sTmIn_D_u8EexvElecStsErr] -> TmDiag/150
  [sTmIn_D_u8EexvBlkErr] -> TmDiag/151
  [sTmIn_D_u8EexvOvrTrvlErr] -> TmDiag/152
  [sTmIn_D_u8EexvNVMFlt] -> TmDiag/153
  [yTmIn_B_EExvPosn2FReq] -> TmDiag/154
  [sTmIn_X_s32EExvPosnReq2F] -> TmDiag/155
  [yTmIn_B_EExvMoveEna2FReq] -> TmDiag/156
  [yTmIn_B_EExvMoveEnaReq2F] -> TmDiag/157
  [yTmIn_B_EExvCal2FReq] -> TmDiag/158
  [yTmIn_B_EExvCalReq2F] -> TmDiag/159
  [sTmIn_D_u8VcEvBexvIniFail] -> TmDiag/160
  [sTmIn_D_u8VcEvBexvOvrTempErr] -> TmDiag/161
  [sTmIn_D_u8VcEvBexvBlkErr] -> TmDiag/162
  [sTmIn_D_u8VcEvBexvErrResp] -> TmDiag/163
  [sTmIn_D_u8VcEvBexvVoltgRangErr] -> TmDiag/164
  [sTmIn_D_u8VcEvBexvNVMFlt] -> TmDiag/165
  [sTmIn_D_u8VcEvCexvIniFail] -> TmDiag/166
  [sTmIn_D_u8VcEvCexvOvrTempErr] -> TmDiag/167
  [sTmIn_D_u8VcEvCexvBlkErr] -> TmDiag/168
  [sTmIn_D_u8VcEvCexvErrResp] -> TmDiag/169
  [sTmIn_D_u8VcEvCexvVoltgRangErr] -> TmDiag/170
  [sTmIn_D_u8VcEvCexvNVMFlt] -> TmDiag/171
  [yTmIn_B_ElAcEnable] -> TmDiag/172
  [sTmIn_D_u8HVoltResonanceStat] -> TmDiag/173
  [sTmIn_D_u8InCurrOverCurrStat] -> TmDiag/174
  [sTmIn_D_u8OverPowerStat] -> TmDiag/175
  [sTmIn_D_u8MotorCurrOverCurrStat] -> TmDiag/176
  [sTmIn_D_u8OverMotorCurrStat] -> TmDiag/177
  [sTmIn_D_u8CmprRotorLockStat] -> TmDiag/178
  [sTmIn_D_u8LiquidSluggingStat] -> TmDiag/179
  [sTmIn_D_u8CmprRAMFault] -> TmDiag/180
  [sTmIn_D_u8CmprROMFault] -> TmDiag/181
  [yTmIn_B_CmprSpd2FReq] -> TmDiag/182
  [sTmIn_n_s32CmprSpdReq2F] -> TmDiag/183
  [yTmIn_B_CmprPwrEna2FReq] -> TmDiag/184
  [sTmIn_Pw_s32CmprPwrEnaReq2F] -> TmDiag/185
  [yTmIn_B_CmprStsEna2FReq] -> TmDiag/186
  [sTmIn_D_u8CmprStsEnaReq2F] -> TmDiag/187
  [sTmIn_D_u8GrlShttrStsShttrTErr] -> TmDiag/188
  [sTmIn_D_u8GrlShttrStsShttrULoErr] -> TmDiag/189
  [sTmIn_D_u8GrlShttrOverVolt] -> TmDiag/190
  [sTmIn_D_u8GrlShttrStsShttrActrFlt] -> TmDiag/191
  [sTmIn_D_u8GrlShttrOvertravelErr] -> TmDiag/192
  [sTmIn_D_u8GrlShttrStsShttrBlkd] -> TmDiag/193
  [sTmIn_D_u8GrlShttrStsShttrSnsrFlt] -> TmDiag/194
  [sTmIn_D_u8GrlShttrStsShttrElecErr] -> TmDiag/195
  [sTmIn_D_u8GrlShttrNVMFlt] -> TmDiag/196
  [yTmIn_B_VaneCalEnbl2FReq] -> TmDiag/197
  [yTmIn_B_VaneCalEnbl2F] -> TmDiag/198
  [yTmIn_B_GrlShttrTrqBst2FReq] -> TmDiag/199
  [sTmIn_D_u8GrlShttrTrqBstReq2F] -> TmDiag/200
  [yTmIn_B_VaneCtrlAngle2FReq] -> TmDiag/201
  [sTmIn_Z_s32VaneCtrlAngleReq2F] -> TmDiag/202
  [yTmIn_B_HvCooltHeatrEnad] -> TmDiag/203
  [sTmIn_D_u8CooltTInSnsrFlt] -> TmDiag/204
  [sTmIn_D_u8CooltTOutSnsrFlt] -> TmDiag/205
  [sTmIn_D_u8TInMtrlSnsrFlt] -> TmDiag/206
  [sTmIn_D_u8SelfTmpSigOvrheatg] -> TmDiag/207
  [sTmIn_D_u8CooltTOutOfRng] -> TmDiag/208
  [sTmIn_D_u8SrvRqrd] -> TmDiag/209
  [sTmIn_D_u8SelfTmpSigHwProtn] -> TmDiag/210
  [sTmIn_D_u8TmpSigProtnOfSelfTmp] -> TmDiag/211
  [sTmIn_D_u8CircForDrvrShoOrOpen] -> TmDiag/212
  [sTmIn_D_u8ULoOutOfRng] -> TmDiag/213
  [sTmIn_D_u8HvOutOfRng] -> TmDiag/214
  [sTmIn_D_u8ICnsOutOfRng] -> TmDiag/215
  [sTmIn_D_u8MemErr] -> TmDiag/216
  [yTmIn_B_PtcT2FReq] -> TmDiag/217
  [sTmIn_Te_s32PtcTReq2F] -> TmDiag/218
  [yTmIn_B_PtcPwr2FReq] -> TmDiag/219
  [sTmIn_Pw_s32PtcPwrReq2F] -> TmDiag/220
  [yTmIn_B_PtcEna2FReq] -> TmDiag/221
  [yTmIn_B_PtcEnaReq2F] -> TmDiag/222
  [yTmIn_B_PtcFlow2FReq] -> TmDiag/223
  [sTmIn_L_s32PtcFlowReq2F] -> TmDiag/224
  [yTmComprCtrl_B_CompOnReq] -> TmDiag/225
  [sTmIn_Te_s32HvBattCooltT] -> TmDiag/226
  [sTmIn_md_s32HvacAirMFlowEstimd] -> TmDiag/227
  [sTmIn_v_s32VehSpdLgt] -> TmDiag/228
  [yTmIn_B_TeEvap] -> TmDiag/229
  [yTmIn_B_EvaprTFrntUD] -> TmDiag/230
  [sTmSigProces_D_u8AdcuConfig] -> TmDiag/231
  [sTmIn_D_u8ShutterConfig] -> TmDiag/232
  [yTmHvchCtrl_B_HpcPtcEnad] -> TmDiag/233
  [sTmIn_D_u8BattCntct] -> TmDiag/234
  [sTmIn_U_s32HvBattUDc] -> TmDiag/235
  [sTmIn_D_u8HvUSplyErrSts] -> TmDiag/236
  [yTmIn_B_AmbTEstimdQf] -> TmDiag/237
  [sTmIn_Te_s32AmbTEstimd] -> TmDiag/238
  [yTmIn_B_AirCondEnbl] -> TmDiag/239
  [sTmIn_D_u8VcEvEexvIniFail] -> TmDiag/240
  [sTmIn_D_u8VcEvEexvOvrTempErr] -> TmDiag/241
  [sTmIn_D_u8VcEvEexvBlkErr] -> TmDiag/242
  [sTmIn_D_u8VcEvEexvErrResp] -> TmDiag/243
  [sTmIn_D_u8VcEvEexvVoltgRangErr] -> TmDiag/244
  [sTmIn_D_u8VcEvEexvNVMFlt] -> TmDiag/245
  [sTmIn_D_u8VcEvBctvOthrErr] -> TmDiag/246
  [sTmIn_D_u8VcEvFltTemBCTV] -> TmDiag/247
  [sTmIn_D_u8VcEvBctvBlk] -> TmDiag/248
  [sTmIn_D_u8VcEvBctvErrResp] -> TmDiag/249
  [sTmIn_D_u8VcEvFltVolBCTV] -> TmDiag/250
  [sTmIn_D_u8VcEvBctvNVMFlt] -> TmDiag/251
  [sTmIn_D_u8VcEvBctvIniFail] -> TmDiag/252
  [sTmIn_D_u8VcEvBcfvOthrErr] -> TmDiag/253
  [sTmIn_D_u8VcEvFltTempBCFV] -> TmDiag/254
  [sTmIn_D_u8VcEvBcfvBlk] -> TmDiag/255
  [sTmIn_D_u8VcEvBcfvErrResp] -> TmDiag/256
  [sTmIn_D_u8VcEvFltVolBCFV] -> TmDiag/257
  [sTmIn_D_u8VcEvBcfvNVMFlt] -> TmDiag/258
  [sTmIn_D_u8VcEvBcfvIniFail] -> TmDiag/259
  [sTmIn_D_u8VcEvEctvDrvMotorFlt] -> TmDiag/260
  [sTmIn_D_u8VcEvWarnECRV] -> TmDiag/261
  [sTmIn_D_u8VcEvFltVolECRV] -> TmDiag/262
  [sTmIn_D_u8VcEvEcrvErrResp] -> TmDiag/263
  [sTmIn_D_u8VcEvAccmUSplyErr] -> TmDiag/264
  [sTmIn_D_u8VcEvAccmOCFlt] -> TmDiag/265
  [sTmIn_D_u8VcEvAccmMotOvrCur] -> TmDiag/266
  [sTmIn_D_u8VcEvAccmComFlt] -> TmDiag/267
  [sTmIn_D_u8VcEvCurDrCirtACCM] -> TmDiag/268
  [sTmIn_D_u8VcEvAccmRotorLock] -> TmDiag/269
  [sTmIn_D_u8VcEvAccmOPFlt] -> TmDiag/270
  [sTmIn_D_u8VcEvLiquidSluggingACCM] -> TmDiag/271
  [sTmIn_D_u8VcEvMemFltAccm] -> TmDiag/272
  [sTmIn_D_u8VcEvTM_AGM_OVRTEMP] -> TmDiag/273
  [sTmIn_D_u8VcEvAgsBlk] -> TmDiag/274
  [sTmIn_D_u8VcEvAgsErrResp] -> TmDiag/275
  [sTmIn_D_u8VcEvAgsVoltErr] -> TmDiag/276
  [sTmIn_D_u8VcEvAgsMechErr] -> TmDiag/277
  [sTmIn_D_u8VcEvAgsNVMFlt] -> TmDiag/278
  [sTmIn_D_u8VcEvAgsElecErr] -> TmDiag/279
  [yTmIn_B_Sov1SGTF] -> TmDiag/280
  [yTmIn_B_Sov1SGflg] -> TmDiag/281
  [sTmIn_D_u8VcEvSov1OP] -> TmDiag/282
  [sTmIn_D_u8VcEvSov1SB] -> TmDiag/283
  [sTmIn_D_u8VcEvSov1SG] -> TmDiag/284
  [sTmIn_D_u8VcEvSGEmotor] -> TmDiag/285
  [sTmIn_D_u8VcEvSBEmotor] -> TmDiag/286
  [sTmIn_D_u8VcEvOCEmotor] -> TmDiag/287
  [sTmIn_D_u8VcEvEmPmpOvrTShutDwn] -> TmDiag/288
  [sTmIn_D_u8VcEvEmPmpStall] -> TmDiag/289
  [sTmIn_D_u8VcEvEmPmpVolErr] -> TmDiag/290
  [sTmIn_D_u8VcEvEmPmpDyRn] -> TmDiag/291
  [sTmIn_D_u8VcEvSGBatteryPmp] -> TmDiag/292
  [sTmIn_D_u8VcEvSBBatteryPmp] -> TmDiag/293
  [sTmIn_D_u8VcEvOCBatteryPmp] -> TmDiag/294
  [yTmIn_B_Sov2SGTF] -> TmDiag/295
  [yTmIn_B_Sov2SGflg] -> TmDiag/296
  [sTmIn_D_u8VcEvSov2OP] -> TmDiag/297
  [sTmIn_D_u8VcEvSov2SB] -> TmDiag/298
  [sTmIn_D_u8VcEvSov2SG] -> TmDiag/299
  [yTmIn_B_Sov3SGTF] -> TmDiag/300
  [yTmIn_B_Sov3SGflg] -> TmDiag/301
  [sTmIn_D_u8VcEvSov3OP] -> TmDiag/302
  [sTmIn_D_u8VcEvSov3SB] -> TmDiag/303
  [sTmIn_D_u8VcEvSov3SG] -> TmDiag/304
  [yTmIn_B_Sov4SGTF] -> TmDiag/305
  [yTmIn_B_Sov4SGflg] -> TmDiag/306
  [sTmIn_D_u8VcEvSov4OP] -> TmDiag/307
  [sTmIn_D_u8VcEvSov4SB] -> TmDiag/308
  [sTmIn_D_u8VcEvSov4SG] -> TmDiag/309
  [yTmIn_B_Sov5SGTF] -> TmDiag/310
  [yTmIn_B_Sov5SGflg] -> TmDiag/311
  [sTmIn_D_u8VcEvSov5OP] -> TmDiag/312
  [sTmIn_D_u8VcEvSov5SB] -> TmDiag/313
  [sTmIn_D_u8VcEvSov5SG] -> TmDiag/314
  [sTmIn_D_u8VcEvOPFan] -> TmDiag/315
  [sTmIn_D_u8VcEvSGFan] -> TmDiag/316
  [sTmIn_D_u8VcEvFanOvrTShDwn] -> TmDiag/317
  [sTmIn_D_u8VcEvBlokFan] -> TmDiag/318
  [sTmIn_D_u8VcEvVolErrFan] -> TmDiag/319
  [sTmIn_D_u8VcEvCircutInteFlt] -> TmDiag/320
  [sTmIn_D_u8VcEvHmPumpSG] -> TmDiag/321
  [sTmIn_D_u8VcEvHmPumpSB] -> TmDiag/322
  [sTmIn_D_u8VcEvHmPumpOC] -> TmDiag/323
  [sTmIn_D_u8VcEvHmPmpOvrTShutDwn] -> TmDiag/324
  [sTmIn_D_u8VcEvHmPmpStall] -> TmDiag/325
  [sTmIn_D_u8VcEvHmPmpVolErr] -> TmDiag/326
  [sTmIn_D_u8VcEvHmPmpDyRn] -> TmDiag/327
  [sTmIn_D_u8VcEvBattPmpOvrTShutDwn] -> TmDiag/328
  [sTmIn_D_u8VcEvBattPmpStall] -> TmDiag/329
  [sTmIn_D_u8VcEvBattPmpVolErr] -> TmDiag/330
  [sTmIn_D_u8VcEvBattPmpDyn] -> TmDiag/331
  [sTmIn_D_u8VcEvLoSidePOP] -> TmDiag/332
  [sTmIn_D_u8VcEvLoSidePSB] -> TmDiag/333
  [sTmIn_D_u8VcEvHiSidePOP] -> TmDiag/334
  [sTmIn_D_u8VcEvHiSidePSB] -> TmDiag/335
  [sTmIn_D_u8VcEvHiSideTmpSnrSG] -> TmDiag/336
  [sTmIn_D_u8VcEvOutrCondOutTOP] -> TmDiag/337
  [sTmIn_D_u8VcEvChillerOutTSG] -> TmDiag/338
  [sTmIn_D_u8VcEvChillerOutTOP] -> TmDiag/339
  [sTmIn_D_u8VcEvInrCondOutTSG] -> TmDiag/340
  [sTmIn_D_u8VcEvInrCondOutTOP] -> TmDiag/341
  [sTmIn_D_u8VcEvEvapOutTSG] -> TmDiag/342
  [sTmIn_D_u8VcEvEvapOutTOP] -> TmDiag/343
  [sTmIn_D_u8VcEvCmprDischrgTSG] -> TmDiag/344
  [sTmIn_D_u8VcEvCmprDischrgTOP] -> TmDiag/345
  [sTmIn_D_u8VcEvTmpClSrSG] -> TmDiag/346
  [sTmIn_D_u8VcEvTmpClSrOP] -> TmDiag/347
  [sTmIn_D_u8VcEvBattCooltLvlLo] -> TmDiag/348
  [sTmIn_D_u8VcEvNoHpHighSidePSnrOP] -> TmDiag/349
  [sTmIn_D_u8VcEvNoHpHighSidePSnrSB] -> TmDiag/350
  [yTmIn_B_HvacHexAirTQf] -> TmDiag/351
  [yTmIn_B_HvacHexAirTUD] -> TmDiag/352
  [sTmIn_D_u8VcEvIGBTSpOrOpHVCH] -> TmDiag/353
  [sTmIn_D_u8VcEvLoVoOvrHVCH] -> TmDiag/354
  [sTmIn_D_u8VcEvVolMemErrHVCH] -> TmDiag/355
  [sTmIn_D_u8VcEvComFltHVCH] -> TmDiag/356
  [sTmIn_D_u8VcEvHiVoOvrHVCH] -> TmDiag/357
  [sTmIn_D_u8VcEvCoolTempOutOfRng] -> TmDiag/358
  [sTmIn_D_u8VcEvTempSerIntHVCH] -> TmDiag/359
  [sTmIn_D_u8VcEvTempSerOutHVCH] -> TmDiag/360
  [sTmIn_D_u8VcEvHWProtHVCH] -> TmDiag/361
  [sTmIn_D_u8VcEvInterSerTempHVCH] -> TmDiag/362
  [sTmIn_D_u8VcEvCurrOutOfRng] -> TmDiag/363
  [yTmIn_B_GrlShttrAutoCalibReq2FReq] -> TmDiag/364
  [yTmIn_B_GrlShttrAutoCalibReqReq2F] -> TmDiag/365
  [sTmSigProces_p_s32HpAcHiSidePToOut] -> TmDiag/366
  [sTmSigProces_p_s32HiSidePNHPToOut] -> TmDiag/367
  [sTmSigProces_Te_s32MotorCoolt] -> TmDiag/368
  [yTmIn_B_HvacHeatgReq] -> TmDiag/369
  [sTmIn_D_u8HvBattThermReq] -> TmDiag/370
  [sTmIn_D_u8LackRefrigerant] -> TmDiag/371
  [yTmIn_B_MessMissBctv] -> TmDiag/372
  [yTmIn_B_MessMissBCFV] -> TmDiag/373
  [yTmIn_B_MessMissECRV] -> TmDiag/374
  [yTmIn_B_MessMissBEXV] -> TmDiag/375
  [yTmIn_B_MessMissCEXV] -> TmDiag/376
  [yTmIn_B_MessMissEEXV] -> TmDiag/377
  [yTmIn_B_MessMissAccm] -> TmDiag/378
  [yTmIn_B_MessMissAGM] -> TmDiag/379
  [yTmIn_B_MessMissHVCH] -> TmDiag/380
  [sTmIn_Te_s32HvBattCooltTOut] -> TmDiag/381
  [sTmIn_D_u8VcEvEctvBlk] -> TmDiag/382
  [sTmIn_D_u8AccmLoUSplyErrSts] -> TmDiag/383
  [sTmIn_D_u8AccmDrvrSircSnErrStsts] -> TmDiag/384
  [sTmIn_D_u8AccmHvSnsrU1ErrSts] -> TmDiag/385
  [sTmIn_D_u8AccmHvSnsrU2ErrSts] -> TmDiag/386
  [sTmIn_D_u8AccmPhaseWireErrSts] -> TmDiag/387
  [sTmIn_D_u8AccmT1ErrSts] -> TmDiag/388
  [sTmIn_D_u8AccmT2ErrSts] -> TmDiag/389
  [sTmIn_D_u8AccmCmprTOperErr1] -> TmDiag/390
  [sTmIn_D_u8AccmSnsrICrctErrSts] -> TmDiag/391
  [sTmIn_D_u8AccmHvSnsrIErrSts] -> TmDiag/392
  [sTmIn_D_u8AccmCmprTOperErr2] -> TmDiag/393
  [sTmIn_D_u8VcEvOVACCM] -> TmDiag/394
  [sTmIn_D_u8VcEvAccmIgbtOvrTErr] -> TmDiag/395
  [sTmIn_D_u8VcEvAccmSnsrFlt] -> TmDiag/396
  [sTmIn_D_u8VcEvAccmPhaseFail] -> TmDiag/397
  [sTmIn_D_u8VcEvOvrTempHVCH] -> TmDiag/398
  [yTmIn_B_AD4CoolReqForBkpUD] -> TmDiag/399
  [yTmIn_B_AD4CoolReqUD] -> TmDiag/400
  [yTmIn_B_AD4CooltFlowReqForBkpUD] -> TmDiag/401
  [yTmIn_B_AD4CooltFlowReqUD] -> TmDiag/402
  [sTmIn_D_u8ErrRespACCM] -> TmDiag/403
  [yTmIn_B_ErrRespHVCH] -> TmDiag/404
  [sTmIn_D_u8FltInComHVCH] -> TmDiag/405
  [sTmIn_B_HvBattLimnIndcnUD] -> TmDiag/406
  [sTmSigProces_D_u8HvBoostModConfig] -> TmDiag/407
  [sTmEnergyMgr_Pw_s32HPCoolPACCM] -> TmDiag/408
  [sTmEnergyMgr_Pw_s32BattCoolPACCM] -> TmDiag/409
  [sTmEnergyMgr_Pw_s32HvCoolgPwrCns] -> TmDiag/410
  [sTmIn_n_s32ElacCmprActl] -> TmDiag/411
  [sTmSigProces_p_s32LoSideToOut] -> TmDiag/412
  [sTmEnergyMgr_Pw_s32HPHeatPACCM] -> TmDiag/413
  TmDiag/1 -> [yTmDiag_B_SnrDiagEna]
  TmDiag/2 -> [yTmDiag_B_HWActrDiagEna]
  TmDiag/3 -> [yTmDiag_B_LINActrDiagEna]
  TmDiag/4 -> [yTmDiag_B_Diag2FEna]
  TmDiag/5 -> [sTmDiag_D_u8RefriSysFltSt]
  TmDiag/6 -> [sTmDiag_D_u8ClntSysFltSt]
  TmDiag/7 -> [sTmDiag_D_u8VcEvLowSidePSnrOP]
  TmDiag/8 -> [sTmDiag_D_u8LoSidePFltSt]
  TmDiag/9 -> [sTmDiag_D_u8VcEvHiSidePSnrOP]
  TmDiag/10 -> [sTmDiag_D_u8HiSidePFltSt]
  TmDiag/11 -> [sTmDiag_D_u8VcEvHiSideTmpSnrSG]
  TmDiag/12 -> [sTmDiag_D_u8OutrCondOutTFltSt]
  TmDiag/13 -> [sTmDiag_D_u8VcEvChillerOutTSG]
  TmDiag/14 -> [sTmDiag_D_u8ChillerOutTFltSt]
  TmDiag/15 -> [sTmDiag_D_u8VcEvInrCondOutTSG]
  TmDiag/16 -> [sTmDiag_D_u8InrCondOutTFltSt]
  TmDiag/17 -> [sTmDiag_D_u8VcEvEvapOutTSG]
  TmDiag/18 -> [sTmDiag_D_u8EvapOutTFltSt]
  TmDiag/19 -> [sTmDiag_D_u8CmprDischrgTFltSt]
  TmDiag/20 -> [sTmDiag_D_u8ClntTforEmCircFltSt]
  TmDiag/21 -> [sTmDiag_D_u8BattClntLvlFltSt]
  TmDiag/22 -> [sTmDiag_D_u8HiSidePNHPFltSt]
  TmDiag/23 -> [sTmDiag_D_u8Sov1FltSt]
  TmDiag/24 -> [sTmDiag_D_u8Sov2FltSt]
  TmDiag/25 -> [sTmDiag_D_u8HpmSov2Actv2FEnState]
  TmDiag/26 -> [sTmDiag_D_u8Sov3FltSt]
  TmDiag/27 -> [sTmDiag_D_u8HpmSov3Actv2FEnState]
  TmDiag/28 -> [sTmDiag_D_u8Sov4FltSt]
  TmDiag/29 -> [sTmDiag_D_u8ChillerValve2FEnState]
  TmDiag/30 -> [sTmDiag_D_u8Sov5FltSt]
  TmDiag/31 -> [sTmDiag_D_u8EvaprVlvFrnt2FEnState]
  TmDiag/32 -> [sTmDiag_D_u8FanFltSt]
  TmDiag/33 -> [sTmDiag_D_u8FanPwm2FEnState]
  TmDiag/34 -> [sTmDiag_D_u8HmPmpFltSt]
  TmDiag/35 -> [sTmDiag_D_u8PTCPumpSpd2FEnState]
  TmDiag/36 -> [sTmDiag_D_u8BattPmpFltSt]
  TmDiag/37 -> [sTmDiag_D_u8BattCooltPmp2FEnState]
  TmDiag/38 -> [sTmDiag_D_u8EmPmpFltSt]
  TmDiag/39 -> [sTmDiag_D_u8EmCooltPmp2FEnState]
  TmDiag/40 -> [sTmDiag_D_u8BctvFltSt]
  TmDiag/41 -> [sTmDiag_D_u8BctvVlvPos2FEnaState]
  TmDiag/42 -> [sTmDiag_D_u8BctvVlvRef2FEnaState]
  TmDiag/43 -> [sTmDiag_D_u8BcfvFltSt]
  TmDiag/44 -> [sTmDiag_D_u8BcfvVlvPos2FEnaState]
  TmDiag/45 -> [sTmDiag_D_u8BcfvVlvRef2FEnaState]
  TmDiag/46 -> [sTmDiag_D_u8EctvFltSt]
  TmDiag/47 -> [sTmDiag_D_u8EctvVlvPos2FEnaState]
  TmDiag/48 -> [sTmDiag_D_u8EctvVlvMoveEna2FEnaState]
  TmDiag/49 -> [sTmDiag_D_u8BexvFltSt]
  TmDiag/50 -> [sTmDiag_D_u8BexvPosnReq2FEnaState]
  TmDiag/51 -> [sTmDiag_D_u8BexvMoveEna2FEnaState]
  TmDiag/52 -> [sTmDiag_D_u8BexvCal2FEnaState]
  TmDiag/53 -> [sTmDiag_D_u8CexvFltSt]
  TmDiag/54 -> [sTmDiag_D_u8CexvPosnReq2FEnaState]
  TmDiag/55 -> [sTmDiag_D_u8CexvMoveEna2FEnaState]
  TmDiag/56 -> [sTmDiag_D_u8CexvCal2FEnaState]
  TmDiag/57 -> [sTmDiag_D_u8EexvFltSt]
  TmDiag/58 -> [sTmDiag_D_u8EexvPosnReq2FEnaState]
  TmDiag/59 -> [sTmDiag_D_u8EexvMoveEna2FEnaState]
  TmDiag/60 -> [sTmDiag_D_u8EexvCal2FEnaState]
  TmDiag/61 -> [sTmDiag_D_u8AccmFltSt]
  TmDiag/62 -> [sTmDiag_D_u8CmprSpdEna2FEnaState]
  TmDiag/63 -> [sTmDiag_D_u8CmprPwrEna2FEnaState]
  TmDiag/64 -> [sTmDiag_D_u8CmprStsEna2FEnaState]
  TmDiag/65 -> [sTmDiag_D_u8AgmFltSt]
  TmDiag/66 -> [sTmDiag_D_u8VaneCalEnbl2FEnState]
  TmDiag/67 -> [sTmDiag_D_u8GrlShttrTrqBst2FEnState]
  TmDiag/68 -> [sTmDiag_D_u8VaneCtrlAngle2FEnState]
  TmDiag/69 -> [sTmDiag_D_u8HvchFltSt]
  TmDiag/70 -> [sTmDiag_D_u8PtcT2FEnaState]
  TmDiag/71 -> [sTmDiag_D_u8PtcPwr2FEnaState]
  TmDiag/72 -> [sTmDiag_D_u8PtcEna2FEnaState]
  TmDiag/73 -> [sTmDiag_D_u8VcEvLowSidePSnrSB]
  TmDiag/74 -> [sTmDiag_D_u8VcEvHiSidePSnrSB]
  TmDiag/75 -> [sTmDiag_D_u8VcEvChillerOutTOP]
  TmDiag/76 -> [sTmDiag_D_u8VcEvHiSideTmpSnrOP]
  TmDiag/77 -> [sTmDiag_D_u8VcEvInrCondOutTOP]
  TmDiag/78 -> [sTmDiag_D_u8VcEvEvapOutTOP]
  TmDiag/79 -> [sTmDiag_D_u8HpmSov1Actv2FEnState]
  TmDiag/80 -> [sTmDiag_D_u8VcEvHmPumpSB]
  TmDiag/81 -> [sTmDiag_D_u8VcEvSBBatteryPmp]
  TmDiag/82 -> [sTmDiag_D_u8VcEvOCBatteryPmp]
  TmDiag/83 -> [sTmDiag_D_u8VcEvSBEmotor]
  TmDiag/84 -> [sTmDiag_D_u8VcEvOCEmotor]
  TmDiag/85 -> [yTmDiag_B_CarConfigInvalid]
  TmDiag/86 -> [sTmDiag_D_u8HvBattCooltTFltSt]
  TmDiag/87 -> [sTmDiag_D_u8PtcFlow2FEnaState]
  TmDiag/88 -> [sTmDiag_D_u8RefriMod2FInhitReq]
  TmDiag/89 -> [sTmDiag_D_u8WaterMod2FInhitReq]
  TmDiag/90 -> [sTmDiag_D_u8RefrilackFltSt]
  TmDiag/91 -> [yTmDiag_B_CoolantSystemErr]
  TmDiag/92 -> [yTmDiag_B_ACSystemErr]
  TmDiag/93 -> [sTmDiag_D_u8ThermalSystemRedn]
  TmDiag/94 -> [sTmDiag_D_u32ThermalSystemFault]
  TmDiag/95 -> [sTmDiag_D_u8VcEvCmprDischrgTSG]
  TmDiag/96 -> [sTmDiag_D_u8VcEvCmprDischrgTOP]
  TmDiag/97 -> [sTmDiag_D_u8VcEvClntTforEmCircSG]
  TmDiag/98 -> [sTmDiag_D_u8VcEvClntTforEmCircOP]
  TmDiag/99 -> [sTmDiag_D_u8VcEvBattCooltLvlLo]
  TmDiag/100 -> [sTmDiag_D_u8VcEvNoHpHighSidePSnrOP]
  TmDiag/101 -> [sTmDiag_D_u8VcEvNoHpHighSidePSnrSB]
  TmDiag/102 -> [sTmDiag_D_u8TeEvapFltSt]
  TmDiag/103 -> [sTmDiag_D_u8VcEvSov1SB]
  TmDiag/104 -> [sTmDiag_D_u8HvacHexAirTFltSt]
  TmDiag/105 -> [sTmDiag_D_u8VcEvSov1OP]
  TmDiag/106 -> [sTmDiag_D_u8VcEvSov1SG]
  TmDiag/107 -> [sTmDiag_D_u8VcEvSGEmotor]
  TmDiag/108 -> [sTmDiag_D_u8VcEvEmPmpOvrTShutDwn]
  TmDiag/109 -> [sTmDiag_D_u8VcEvEmPmpVolErr]
  TmDiag/110 -> [sTmDiag_D_u8VcEvEmPmpStall]
  TmDiag/111 -> [sTmDiag_D_u8VcEvEmPmpDyRn]
  TmDiag/112 -> [sTmDiag_D_u8VcEvSov2SB]
  TmDiag/113 -> [sTmDiag_D_u8VcEvSov2OP]
  TmDiag/114 -> [sTmDiag_D_u8VcEvSov2SG]
  TmDiag/115 -> [sTmDiag_D_u8VcEvSov3SB]
  TmDiag/116 -> [sTmDiag_D_u8VcEvSov3OP]
  TmDiag/117 -> [sTmDiag_D_u8VcEvSov3SG]
  TmDiag/118 -> [sTmDiag_D_u8VcEvSov4SB]
  TmDiag/119 -> [sTmDiag_D_u8VcEvSov4OP]
  TmDiag/120 -> [sTmDiag_D_u8VcEvSov4SG]
  TmDiag/121 -> [sTmDiag_D_u8VcEvSov5SB]
  TmDiag/122 -> [sTmDiag_D_u8VcEvSov5SG]
  TmDiag/123 -> [sTmDiag_D_u8VcEvOPFan]
  TmDiag/124 -> [sTmDiag_D_u8VcEvFanOvrTShDwn]
  TmDiag/125 -> [sTmDiag_D_u8VcEvHmPumpOC]
  TmDiag/126 -> [sTmDiag_D_u8VcEvSov5OP]
  TmDiag/127 -> [sTmDiag_D_u8VcEvSGFan]
  TmDiag/128 -> [sTmDiag_D_u8VcEvCircutInteFlt]
  TmDiag/129 -> [sTmDiag_D_u8VcEvHmPumpSG]
  TmDiag/130 -> [sTmDiag_D_u8VcEvHmPmpStall]
  TmDiag/131 -> [sTmDiag_D_u8VcEvSBFan]
  TmDiag/132 -> [sTmDiag_D_u8VcEvVolErrFan]
  TmDiag/133 -> [sTmDiag_D_u8VcEvHmPmpOvrTShutDwn]
  TmDiag/134 -> [sTmDiag_D_u8VcEvSGBatteryPmp]
  TmDiag/135 -> [sTmDiag_D_u8VcEvBattPmpVolErr]
  TmDiag/136 -> [sTmDiag_D_u8VcEvBlokFan]
  TmDiag/137 -> [sTmDiag_D_u8VcEvHmPmpVolErr]
  TmDiag/138 -> [sTmDiag_D_u8VcEvHmPmpDyRn]
  TmDiag/139 -> [sTmDiag_D_u8VcEvBattPmpOvrTShutDwn]
  TmDiag/140 -> [sTmDiag_D_u8VcEvBattPmpStall]
  TmDiag/141 -> [sTmDiag_D_u8VcEvBattPmpDyn]
  TmDiag/142 -> [sTmDiag_D_u8VcEvBexvVoltgRangErr]
  TmDiag/143 -> [sTmDiag_D_u8VcEvBexvIniFail]
  TmDiag/144 -> [sTmDiag_D_u8VcEvCexvOvrTempErr]
  TmDiag/145 -> [sTmDiag_D_u8VcEvEexvBlkErr]
  TmDiag/146 -> [sTmDiag_D_u8VcEvBexvBlkErr]
  TmDiag/147 -> [sTmDiag_D_u8VcEvBexvOvrTempErr]
  TmDiag/148 -> [sTmDiag_D_u8VcEvCexvBlkErr]
  TmDiag/149 -> [sTmDiag_D_u8VcEvEexvIniFail]
  TmDiag/150 -> [sTmDiag_D_u8VcEvBctvNVMFlt]
  TmDiag/151 -> [sTmDiag_D_u8VcEvBexvNVMFlt]
  TmDiag/152 -> [sTmDiag_D_u8VcEvCexvVoltgRangErr]
  TmDiag/153 -> [sTmDiag_D_u8VcEvEexvVoltgRangErr]
  TmDiag/154 -> [sTmDiag_D_u8VcEvEexvNVMFlt]
  TmDiag/155 -> [sTmDiag_D_u8VcEvFltTempBCFV]
  TmDiag/156 -> [sTmDiag_D_u8VcEvCexvIniFail]
  TmDiag/157 -> [sTmDiag_D_u8VcEvCexvNVMFlt]
  TmDiag/158 -> [sTmDiag_D_u8VcEvFltTemBCTV]
  TmDiag/159 -> [sTmDiag_D_u8VcEvBcfvIniFail]
  TmDiag/160 -> [sTmDiag_D_u8VcEvBcfvNVMFlt]
  TmDiag/161 -> [sTmDiag_D_u8VcEvEexvOvrTempErr]
  TmDiag/162 -> [sTmDiag_D_u8VcEvFltVolBCTV]
  TmDiag/163 -> [sTmDiag_D_u8VcEvFltVolBCFV]
  TmDiag/164 -> [sTmDiag_D_u8VcEvFltVolECRV]
  TmDiag/165 -> [sTmDiag_D_u8VcEvOPACCM]
  TmDiag/166 -> [sTmDiag_D_u8VcEvBctvIniFail]
  TmDiag/167 -> [sTmDiag_D_u8VcEvBctvBlk]
  TmDiag/168 -> [sTmDiag_D_u8VcEvWarnECRV]
  TmDiag/169 -> [sTmDiag_D_u8VcEvEctvDrvMotorFlt]
  TmDiag/170 -> [sTmDiag_D_u8VcEvLiquidSluggingACCM]
  TmDiag/171 -> [sTmDiag_D_u8VcEvBctvOthrErr]
  TmDiag/172 -> [sTmDiag_D_u8VcEvBcfvBlk]
  TmDiag/173 -> [sTmDiag_D_u8VcEvOCACCM]
  TmDiag/174 -> [sTmDiag_D_u8VcEvRotorLockACCM]
  TmDiag/175 -> [sTmDiag_D_u8VcEvAgsMechErr]
  TmDiag/176 -> [sTmDiag_D_u8VcEvBcfvOthrErr]
  TmDiag/177 -> [sTmDiag_D_u8VcEvCurMotACCM]
  TmDiag/178 -> [sTmDiag_D_u8VcEvMemFltAccm]
  TmDiag/179 -> [sTmDiag_D_u8VcEvTM_AGM_OVRTEMP]
  TmDiag/180 -> [sTmDiag_D_u8VcEvAgsBlk]
  TmDiag/181 -> [sTmDiag_D_u8VcEvAccmUSplyErr]
  TmDiag/182 -> [sTmDiag_D_u8VcEvCurDrCirtACCM]
  TmDiag/183 -> [sTmDiag_D_u8VcEvAgsVoltErr]
  TmDiag/184 -> [sTmDiag_D_u8VcEvAgsElecErr]
  TmDiag/185 -> [sTmDiag_D_u8VcEvAgsNVMFlt]
  TmDiag/186 -> [sTmDiag_D_u8VcEvTempSerIntHVCH]
  TmDiag/187 -> [sTmDiag_D_u8VcEvTempSerOutHVCH]
  TmDiag/188 -> [sTmDiag_D_u8VcEvInterSerTempHVCH]
  TmDiag/189 -> [sTmDiag_D_u8VcEvOvrTempHVCH]
  TmDiag/190 -> [sTmDiag_D_u8VcEvCoolTempOutOfRng]
  TmDiag/191 -> [sTmDiag_D_u8VcEvHWProtHVCH]
  TmDiag/192 -> [sTmDiag_D_u8VcEvIGBTSpOrOpHVCH]
  TmDiag/193 -> [sTmDiag_D_u8VcEvLoVoOvrHVCH]
  TmDiag/194 -> [sTmDiag_D_u8VcEvHiVoOvrHVCH]
  TmDiag/195 -> [sTmDiag_D_u8VcEvCurrOutOfRng]
  TmDiag/196 -> [sTmDiag_D_u8VcEvVolMemErrHVCH]
  TmDiag/197 -> [sTmDiag_D_u8GrlShttrAutoCalibReq2FEnState]
  TmDiag/198 -> [yTmDiag_B_HpmSov1ActvCmd2F]
  TmDiag/199 -> [yTmDiag_B_HpmSov2ActvCmd2F]
  TmDiag/200 -> [yTmDiag_B_HpmSov3ActvCmd2F]
  TmDiag/201 -> [yTmDiag_B_ChillerValveReq2F]
  TmDiag/202 -> [yTmDiag_B_EvaprVlvReqFrnt2F]
  TmDiag/203 -> [sTmDiag_X_s32FanPwmReq2F]
  TmDiag/204 -> [sTmDiag_X_s32PTCPumpSpdReq2F]
  TmDiag/205 -> [sTmDiag_X_s32BattCooltPmpReq2F]
  TmDiag/206 -> [sTmDiag_X_s32EmCooltPmpReq2F]
  TmDiag/207 -> [sTmDiag_D_u8BctvVlvRefReq2F]
  TmDiag/208 -> [sTmDiag_X_u8EctvVlvPosReq2F]
  TmDiag/209 -> [sTmDiag_X_s32BexvPosnReq2F]
  TmDiag/210 -> [yTmDiag_B_BexvCalReq2F]
  TmDiag/211 -> [yTmDiag_B_CexvMoveEnReq2F]
  TmDiag/212 -> [sTmDiag_X_s32EexvPosnReq2F]
  TmDiag/213 -> [yTmDiag_B_EexvCalReq2F]
  TmDiag/214 -> [sTmDiag_Pw_s32CmprPwrEnaReq2F]
  TmDiag/215 -> [sTmDiag_D_u8CmprStsEnaReq2F]
  TmDiag/216 -> [sTmDiag_X_u8BctvVlvPosReq2F]
  TmDiag/217 -> [sTmDiag_X_u8BcfvVlvPosReq2F]
  TmDiag/218 -> [sTmDiag_D_u8BcfvVlvRefReq2F]
  TmDiag/219 -> [yTmDiag_B_EctvVlvMoveEnaReq2F]
  TmDiag/220 -> [yTmDiag_B_BexvMoveEnReq2F]
  TmDiag/221 -> [sTmDiag_X_s32CexvPosnReq2F]
  TmDiag/222 -> [yTmDiag_B_CexvCalReq2F]
  TmDiag/223 -> [yTmDiag_B_EexvMoveEnReq2F]
  TmDiag/224 -> [sTmDiag_n_s32CmprSpdReq2F]
  TmDiag/225 -> [yTmDiag_B_VaneCalEnbl2F]
  TmDiag/226 -> [sTmDiag_D_u8GrlShttrTrqBstReq2F]
  TmDiag/227 -> [sTmDiag_Z_s32VaneCtrlAngleReq2F]
  TmDiag/228 -> [yTmDiag_B_GrlShttrAutoCalibReqReq2F]
  TmDiag/229 -> [sTmDiag_Te_s32PtcTReq2F]
  TmDiag/230 -> [sTmDiag_Pw_s32PtcPwrReq2F]
  TmDiag/231 -> [yTmDiag_B_PtcEnaReq2F]
  TmDiag/232 -> [sTmDiag_L_s32PtcFlowrateReq2F]
  TmDiag/233 -> [sTmDiag_D_u8LackRefrigerant]
  TmDiag/234 -> [sTmDiag_D_u8HvBattCooltTOutFltSt]
  TmDiag/235 -> [sTmDiag_D_u8VcEvEctvBlk]
  TmDiag/236 -> [sTmDiag_D_u8VcEvOVACCM]
  TmDiag/237 -> [sTmDiag_D_u8VcEvAccmIgbtOvrTErr]
  TmDiag/238 -> [sTmDiag_D_u8VcEvAccmSnsrFlt]
  TmDiag/239 -> [sTmDiag_D_u8VcEvAccmPhaseFail]
  TmDiag/240 -> [yTmDiag_B_AD4CoolReqForBkpUDLost]
  TmDiag/241 -> [yTmDiag_B_AD4CoolReqUDLost]
  TmDiag/242 -> [yTmDiag_B_AD4CooltFlowReqForBkpUDLost]
  TmDiag/243 -> [yTmDiag_B_AD4CooltFlowReqUDLost]
  TmDiag/244 -> [sTmDiag_D_u8VcEvAccmComFlt]
  TmDiag/245 -> [sTmDiag_D_u8VcEvComFltHVCH]
  TmDiag/246 -> [yTmDiag_B_HvBattLimnIndcnUDLost]
  TmDiag/247 -> [sTmDiag_t_s32FanOutSGTLow]
  TmDiag/248 -> [sTmDiag_t_s32HmPumpSGTLow]
  TmDiag/249 -> [sTmDiag_t_s32BattPmpSGTLow]
  TmDiag/250 -> [sTmDiag_t_s32EmotPmpSGTLow]
  TmDiag/251 -> [sTmDiag_D_u8RefriMoreOrLessFltSt]
  TmDiag/252 -> [sTmDiag_t_s32RefriMoreOrLessFltSt]
  TmDiag/253 -> [sTmDiag_Z_u8SystemCurrCOP]
  TmDiag/254 -> [sTmDiag_Z_u8CmpPerfmaCOP]
  [TmAfCtrl_100] -> TmAfCtrl/1
  [yTmIn_B_ImpactDetect] -> TmAfCtrl/2
  [sTmIn_D_u8GrlShttrStsShttrCalActv] -> TmAfCtrl/3
  [sTmIn_D_u8GrlShttrStsShttrCalIndcd] -> TmAfCtrl/4
  [sTmIn_D_u8GrlShttrMoveActive] -> TmAfCtrl/5
  [sTmIn_D_u8GrlHldTrqActive] -> TmAfCtrl/6
  [sTmIn_X_s32GrlShttrStsShttrPosnRaw] -> TmAfCtrl/7
  [sTmIn_D_u8GrlActTrqBoost] -> TmAfCtrl/8
  [sTmColtModeMgr_D_u8WSMReqMode] -> TmAfCtrl/9
  [sTmIn_D_u8HvBattThermReq] -> TmAfCtrl/10
  [sTmSigProces_D_u8PassiveCoolEnFlag] -> TmAfCtrl/11
  [sTmIn_D_u8HvActvSts] -> TmAfCtrl/12
  [sTmIn_D_u8OnBdChrgrHndlSts] -> TmAfCtrl/13
  [sTmIn_D_u8HvActvReq] -> TmAfCtrl/14
  [sTmIn_D_u8PowerPackStatus] -> TmAfCtrl/15
  [sTmIn_D_u8EctvPosSts] -> TmAfCtrl/16
  [sTmColtVlvCtrl_D_u8HpcEctvReq] -> TmAfCtrl/17
  [sTmSigProces_Te_s32MotorDvcCtl] -> TmAfCtrl/18
  [sTmSigProces_Te_s32MotorCoolt] -> TmAfCtrl/19
  [sTmIn_Te_s32EradWndgActl] -> TmAfCtrl/20
  [sTmIn_Te_s32EradInvActl] -> TmAfCtrl/21
  [sTmIn_Te_s32HvgWndgActl] -> TmAfCtrl/22
  [sTmIn_Te_s32HvgInvActl] -> TmAfCtrl/23
  [sTmIn_Te_s32OnBdChrgrCooltT] -> TmAfCtrl/24
  [sTmIn_Te_s32WhlMotSysCooltT] -> TmAfCtrl/25
  [sTmPumpCtrl_X_s32MpumpPwmReq] -> TmAfCtrl/26
  [yTmSigProces_B_LaunchCtrl] -> TmAfCtrl/27
  [sTmIn_Te_s32AmbTEstimd] -> TmAfCtrl/28
  [sTmSigProces_p_u16PHighSideNHP] -> TmAfCtrl/29
  [sTmIn_v_s32VehSpdLgt] -> TmAfCtrl/30
  [sTmIn_D_u8HeatPump] -> TmAfCtrl/31
  [sTmRefriModeMgr_D_u8HpModeCmd] -> TmAfCtrl/32
  [sTmDiag_D_u8HiSidePFltSt] -> TmAfCtrl/33
  [sTmSigProces_Te_s32SatLp] -> TmAfCtrl/34
  [yTmComprCtrl_B_CompOnReq] -> TmAfCtrl/35
  [sTmSigProces_p_u16PHighSide] -> TmAfCtrl/36
  [sTmComprCtrl_n_u16CompRpmReq] -> TmAfCtrl/37
  [sTmRefriModeMgr_D_u8HpFmCmd] -> TmAfCtrl/38
  [sTmIn_X_s32CexvPosSts] -> TmAfCtrl/39
  [sTmDiag_D_u8HiSidePNHPFltSt] -> TmAfCtrl/40
  [sTmRefriModeMgr_D_u8HPCurMode] -> TmAfCtrl/41
  [sTmDiag_D_u8FanFltSt] -> TmAfCtrl/42
  [sTmIn_n_s32ElacCmprActl] -> TmAfCtrl/43
  [sTmIn_D_u8LVPwrSplyErrSts] -> TmAfCtrl/44
  [yTmRefriModeMgr_B_InterChillDeicing] -> TmAfCtrl/45
  [yTmIn_B_ChargePsr] -> TmAfCtrl/46
  [sTmIn_D_u8HvCoolgCmd] -> TmAfCtrl/47
  [sTmIn_D_u8HvHvacCmd] -> TmAfCtrl/48
  [sTmIn_D_u8CarModSts1] -> TmAfCtrl/49
  [sTmIn_D_u8ShutterConfig] -> TmAfCtrl/50
  [sTmDiag_D_u8AgmFltSt] -> TmAfCtrl/51
  [sTmIn_Tq_s32TotAxle] -> TmAfCtrl/52
  [sTmSigProces_D_u16HVvBattLimnIndcn] -> TmAfCtrl/53
  [sTmDiag_D_u8FanPwm2FEnState] -> TmAfCtrl/54
  [sTmDiag_X_s32FanPwmReq2F] -> TmAfCtrl/55
  [sTmDiag_Z_s32VaneCtrlAngleReq2F] -> TmAfCtrl/56
  [sTmDiag_D_u8VaneCtrlAngle2FEnState] -> TmAfCtrl/57
  [yTmDiag_B_GrlShttrAutoCalibReqReq2F] -> TmAfCtrl/58
  [sTmDiag_D_u8GrlShttrAutoCalibReq2FEnState] -> TmAfCtrl/59
  [sTmDiag_D_u8GrlShttrTrqBstReq2F] -> TmAfCtrl/60
  [sTmDiag_D_u8GrlShttrTrqBst2FEnState] -> TmAfCtrl/61
  [sTmIn_D_u8DCChrgSt] -> TmAfCtrl/62
  [sTmIn_D_u8UsgModSts1WdSts] -> TmAfCtrl/63
  TmAfCtrl/1 -> [sTmAfCtrl_md_s32AfPred]
  TmAfCtrl/2 -> [sTmAfCtrl_X_s32FanPwmReq]
  TmAfCtrl/3 -> [yTmAfCtrl_B_PtCoolgPostRunActv]
  TmAfCtrl/4 -> [yTmAfCtrl_B_ShttrNetReq]
  TmAfCtrl/5 -> [sTmAfCtrl_fq_s32FanPwmFrq]
  TmAfCtrl/6 -> [sTmAfCtrl_X_s32VaneCtrlAngleReq]
  TmAfCtrl/7 -> [sTmAfCtrl_D_u8GrlShttrTrqBstReq]
  TmAfCtrl/8 -> [yTmAfCtrl_B_GrlShttrAutoCalibReq]
  TmAfCtrl/9 -> [sTmAfCtrl_md_s32AirFlowReqSeld]
  TmAfCtrl/10 -> [yTmAfCtrl_B_VaneCalEnbl]
